simulink library "outp"  (R2021b)
(part 6 of 7)

  VTPM_S4ID_raw32_Inproc : FVT_lib/outp/OverrideAndLimit  SystemSampleTime=-1  VariantActivationTime=update diagram  Latency=0  AutoFrameSizeCalculation=off
      link override Signal_Limit/_maxval: Value=KOUTP_S4ID_raw32_maxval
      link override Signal_Limit/_minval: Value=KOUTP_S4ID_raw32_minval
      link override Signal_Override/_ovrdflg: Value=KOUTP_S4ID_raw32_ovrdflg
      link override Signal_Override/_ovrdval: Value=KOUTP_S4ID_raw32_ovrdval
  VTPM_S4L_enum_Inproc : FVT_lib/outp/OverrideAndLimit  SystemSampleTime=-1  VariantActivationTime=update diagram  Latency=0  AutoFrameSizeCalculation=off
      link override Signal_Limit/_maxval: Value=KOUTP_S4L_enum_maxval
      link override Signal_Limit/_minval: Value=KOUTP_S4L_enum_minval
      link override Signal_Override/_ovrdflg: Value=KOUTP_S4L_enum_ovrdflg
      link override Signal_Override/_ovrdval: Value=KOUTP_S4L_enum_ovrdval
  VTPM_S4WheelDebugALTU_pct_Inproc : FVT_lib/outp/OverrideAndLimit  SystemSampleTime=-1  VariantActivationTime=update diagram  Latency=0  AutoFrameSizeCalculation=off
      link override Signal_Limit/_maxval: Value=KOUTP_S4WheelDebugALTU_pct_maxval
      link override Signal_Limit/_minval: Value=KOUTP_S4WheelDebugALTU_pct_minval
      link override Signal_Override/_ovrdflg: Value=KOUTP_S4WheelDebugALTU_pct_ovrdflg
      link override Signal_Override/_ovrdval: Value=KOUTP_S4WheelDebugALTU_pct_ovrdval
  VTPM_SetIDLoc_flg_Inproc : FVT_lib/outp/OverrideAndLimit  SystemSampleTime=-1  VariantActivationTime=update diagram  Latency=0  AutoFrameSizeCalculation=off
      link override Signal_Limit/_maxval: Value=KOUTP_SetIDLoc_flg_maxval
      link override Signal_Limit/_minval: Value=KOUTP_SetIDLoc_flg_minval
      link override Signal_Override/_ovrdflg: Value=KOUTP_SetIDLoc_flg_ovrdflg
      link override Signal_Override/_ovrdval: Value=KOUTP_SetIDLoc_flg_ovrdval
  VTPM_TPMSCaliButtAllow_flg_Inproc : FVT_lib/outp/OverrideAndLimit  SystemSampleTime=-1  VariantActivationTime=update diagram  Latency=0  AutoFrameSizeCalculation=off
      link override Signal_Limit/_maxval: Value=KOUTP_TPMSCaliButtAllow_flg_maxval
      link override Signal_Limit/_minval: Value=KOUTP_TPMSCaliButtAllow_flg_minval
      link override Signal_Override/_ovrdflg: Value=KOUTP_TPMSCaliButtAllow_flg_ovrdflg
      link override Signal_Override/_ovrdval: Value=KOUTP_TPMSCaliButtAllow_flg_ovrdval
  VTPM_TPMSResButtAllow_flg_Inproc : FVT_lib/outp/OverrideAndLimit  SystemSampleTime=-1  VariantActivationTime=update diagram  Latency=0  AutoFrameSizeCalculation=off
      link override Signal_Limit/_maxval: Value=KOUTP_TPMSResButtAllow_flg_maxval
      link override Signal_Limit/_minval: Value=KOUTP_TPMSResButtAllow_flg_minval
      link override Signal_Override/_ovrdflg: Value=KOUTP_TPMSResButtAllow_flg_ovrdflg
      link override Signal_Override/_ovrdval: Value=KOUTP_TPMSResButtAllow_flg_ovrdval
  VTPM_TPMSResButt_flg_Inproc : FVT_lib/outp/OverrideAndLimit  SystemSampleTime=-1  VariantActivationTime=update diagram  Latency=0  AutoFrameSizeCalculation=off
      link override Signal_Limit/_maxval: Value=KOUTP_TPMSResButt_flg_maxval
      link override Signal_Limit/_minval: Value=KOUTP_TPMSResButt_flg_minval
      link override Signal_Override/_ovrdflg: Value=KOUTP_TPMSResButt_flg_ovrdflg
      link override Signal_Override/_ovrdval: Value=KOUTP_TPMSResButt_flg_ovrdval
  VTPM_TPMSStorge_flg_Inproc : FVT_lib/outp/OverrideAndLimit  SystemSampleTime=-1  VariantActivationTime=update diagram  Latency=0  AutoFrameSizeCalculation=off
      link override Signal_Limit/_maxval: Value=KOUTP_TPMSStorge_flg_maxval
      link override Signal_Limit/_minval: Value=KOUTP_TPMSStorge_flg_minval
      link override Signal_Override/_ovrdflg: Value=KOUTP_TPMSStorge_flg_ovrdflg
      link override Signal_Override/_ovrdval: Value=KOUTP_TPMSStorge_flg_ovrdval
  VTPM_TPMSWarnIndi_enum_Inproc : FVT_lib/outp/OverrideAndLimit  SystemSampleTime=-1  VariantActivationTime=update diagram  Latency=0  AutoFrameSizeCalculation=off
      link override Signal_Limit/_maxval: Value=KOUTP_TPMSWarnIndi_enum_maxval
      link override Signal_Limit/_minval: Value=KOUTP_TPMSWarnIndi_enum_minval
      link override Signal_Override/_ovrdflg: Value=KOUTP_TPMSWarnIndi_enum_ovrdflg
      link override Signal_Override/_ovrdval: Value=KOUTP_TPMSWarnIndi_enum_ovrdval
  VTPM_WriteChkLFID_raw_Inproc : FVT_lib/outp/OverrideAndLimit  SystemSampleTime=-1  VariantActivationTime=update diagram  Latency=0  AutoFrameSizeCalculation=off
      link override Signal_Limit/_maxval: Value=KOUTP_WriteChkLFID_raw_maxval
      link override Signal_Limit/_minval: Value=KOUTP_WriteChkLFID_raw_minval
      link override Signal_Override/_ovrdflg: Value=KOUTP_WriteChkLFID_raw_ovrdflg
      link override Signal_Override/_ovrdval: Value=KOUTP_WriteChkLFID_raw_ovrdval
  VTPM_WriteChkLRID_raw_Inproc : FVT_lib/outp/OverrideAndLimit  SystemSampleTime=-1  VariantActivationTime=update diagram  Latency=0  AutoFrameSizeCalculation=off
      link override Signal_Limit/_maxval: Value=KOUTP_WriteChkLRID_raw_maxval
      link override Signal_Limit/_minval: Value=KOUTP_WriteChkLRID_raw_minval
      link override Signal_Override/_ovrdflg: Value=KOUTP_WriteChkLRID_raw_ovrdflg
      link override Signal_Override/_ovrdval: Value=KOUTP_WriteChkLRID_raw_ovrdval
  VTPM_WriteChkRFID_raw_Inproc : FVT_lib/outp/OverrideAndLimit  SystemSampleTime=-1  VariantActivationTime=update diagram  Latency=0  AutoFrameSizeCalculation=off
      link override Signal_Limit/_maxval: Value=KOUTP_WriteChkRFID_raw_maxval
      link override Signal_Limit/_minval: Value=KOUTP_WriteChkRFID_raw_minval
      link override Signal_Override/_ovrdflg: Value=KOUTP_WriteChkRFID_raw_ovrdflg
      link override Signal_Override/_ovrdval: Value=KOUTP_WriteChkRFID_raw_ovrdval
  VTPM_WriteChkRRID_raw_Inproc : FVT_lib/outp/OverrideAndLimit  SystemSampleTime=-1  VariantActivationTime=update diagram  Latency=0  AutoFrameSizeCalculation=off
      link override Signal_Limit/_maxval: Value=KOUTP_WriteChkRRID_raw_maxval
      link override Signal_Limit/_minval: Value=KOUTP_WriteChkRRID_raw_minval
      link override Signal_Override/_ovrdflg: Value=KOUTP_WriteChkRRID_raw_ovrdflg
      link override Signal_Override/_ovrdval: Value=KOUTP_WriteChkRRID_raw_ovrdval
  VTPM_WriteChkfinLFID_raw_Inproc : FVT_lib/outp/OverrideAndLimit  SystemSampleTime=-1  VariantActivationTime=update diagram  Latency=0  AutoFrameSizeCalculation=off
      link override Signal_Limit/_maxval: Value=KOUTP_WriteChkfinLFID_raw_maxval
      link override Signal_Limit/_minval: Value=KOUTP_WriteChkfinLFID_raw_minval
      link override Signal_Override/_ovrdflg: Value=KOUTP_WriteChkfinLFID_raw_ovrdflg
      link override Signal_Override/_ovrdval: Value=KOUTP_WriteChkfinLFID_raw_ovrdval
  VTPM_WriteChkfinLRID_raw_Inproc : FVT_lib/outp/OverrideAndLimit  SystemSampleTime=-1  VariantActivationTime=update diagram  Latency=0  AutoFrameSizeCalculation=off
      link override Signal_Limit/_maxval: Value=KOUTP_WriteChkfinLRID_raw_maxval
      link override Signal_Limit/_minval: Value=KOUTP_WriteChkfinLRID_raw_minval
      link override Signal_Override/_ovrdflg: Value=KOUTP_WriteChkfinLRID_raw_ovrdflg
      link override Signal_Override/_ovrdval: Value=KOUTP_WriteChkfinLRID_raw_ovrdval
  VTPM_WriteChkfinRFID_raw_Inproc : FVT_lib/outp/OverrideAndLimit  SystemSampleTime=-1  VariantActivationTime=update diagram  Latency=0  AutoFrameSizeCalculation=off
      link override Signal_Limit/_maxval: Value=KOUTP_WriteChkfinRFID_raw_maxval
      link override Signal_Limit/_minval: Value=KOUTP_WriteChkfinRFID_raw_minval
      link override Signal_Override/_ovrdflg: Value=KOUTP_WriteChkfinRFID_raw_ovrdflg
      link override Signal_Override/_ovrdval: Value=KOUTP_WriteChkfinRFID_raw_ovrdval
  VTPM_WriteChkfinRRID_raw_Inproc : FVT_lib/outp/OverrideAndLimit  SystemSampleTime=-1  VariantActivationTime=update diagram  Latency=0  AutoFrameSizeCalculation=off
      link override Signal_Limit/_maxval: Value=KOUTP_WriteChkfinRRID_raw_maxval
      link override Signal_Limit/_minval: Value=KOUTP_WriteChkfinRRID_raw_minval
      link override Signal_Override/_ovrdflg: Value=KOUTP_WriteChkfinRRID_raw_ovrdflg
      link override Signal_Override/_ovrdval: Value=KOUTP_WriteChkfinRRID_raw_ovrdval
  VTPM_unlearnSfailvalid_enum_Inproc : FVT_lib/outp/OverrideAndLimit  SystemSampleTime=-1  VariantActivationTime=update diagram  Latency=0  AutoFrameSizeCalculation=off
      link override Signal_Limit/_maxval: Value=KOUTP_unlearnSfailvalid_enum_maxval
      link override Signal_Limit/_minval: Value=KOUTP_unlearnSfailvalid_enum_minval
      link override Signal_Override/_ovrdflg: Value=KOUTP_unlearnSfailvalid_enum_ovrdflg
      link override Signal_Override/_ovrdval: Value=KOUTP_unlearnSfailvalid_enum_ovrdval
  VTPM_unlearnSfali_flg_Inproc : FVT_lib/outp/OverrideAndLimit  SystemSampleTime=-1  VariantActivationTime=update diagram  Latency=0  AutoFrameSizeCalculation=off
      link override Signal_Limit/_maxval: Value=KOUTP_unlearnSfali_flg_maxval
      link override Signal_Limit/_minval: Value=KOUTP_unlearnSfali_flg_minval
      link override Signal_Override/_ovrdflg: Value=KOUTP_unlearnSfali_flg_ovrdflg
      link override Signal_Override/_ovrdval: Value=KOUTP_unlearnSfali_flg_ovrdval
  VTQD_ActParkRequest_flg_Inproc : FVT_lib/outp/OverrideAndLimit  SystemSampleTime=-1  VariantActivationTime=update diagram  Latency=0  AutoFrameSizeCalculation=off
      link override Signal_Limit/_maxval: Value=KOUTP_ActParkRequest_flg_maxval
      link override Signal_Limit/_minval: Value=KOUTP_ActParkRequest_flg_minval
      link override Signal_Override/_ovrdflg: Value=KOUTP_ActParkRequest_flg_ovrdflg
      link override Signal_Override/_ovrdval: Value=KOUTP_ActParkRequest_flg_ovrdval
  VTQD_CreepON_flg_Inproc : FVT_lib/outp/OverrideAndLimit  SystemSampleTime=-1  VariantActivationTime=update diagram  Latency=0  AutoFrameSizeCalculation=off
      link override Signal_Limit/_maxval: Value=KOUTP_CreepON_flg_maxval
      link override Signal_Limit/_minval: Value=KOUTP_CreepON_flg_minval
      link override Signal_Override/_ovrdflg: Value=KOUTP_CreepON_flg_ovrdflg
      link override Signal_Override/_ovrdval: Value=KOUTP_CreepON_flg_ovrdval
  VTQD_DriveProtEn_flg_Inproc : FVT_lib/outp/OverrideAndLimit  SystemSampleTime=-1  VariantActivationTime=update diagram  Latency=0  AutoFrameSizeCalculation=off
      link override Signal_Limit/_maxval: Value=KOUTP_DriveProtEn_flg_maxval
      link override Signal_Limit/_minval: Value=KOUTP_DriveProtEn_flg_minval
      link override Signal_Override/_ovrdflg: Value=KOUTP_DriveProtEn_flg_ovrdflg
      link override Signal_Override/_ovrdval: Value=KOUTP_DriveProtEn_flg_ovrdval
  VTQD_DriverWhlTqDemFr_Nm_Inproc : FVT_lib/outp/OverrideAndLimit  SystemSampleTime=-1  VariantActivationTime=update diagram  Latency=0  AutoFrameSizeCalculation=off
      link override Signal_Limit/_maxval: Value=KOUTP_DriverWhlTqDemFr_Nm_maxval
      link override Signal_Limit/_minval: Value=KOUTP_DriverWhlTqDemFr_Nm_minval
      link override Signal_Override/_ovrdflg: Value=KOUTP_DriverWhlTqDemFr_Nm_ovrdflg
      link override Signal_Override/_ovrdval: Value=KOUTP_DriverWhlTqDemFr_Nm_ovrdval
  VTQD_DriverWhlTqDemRr_Nm_Inproc : FVT_lib/outp/OverrideAndLimit  SystemSampleTime=-1  VariantActivationTime=update diagram  Latency=0  AutoFrameSizeCalculation=off
      link override Signal_Limit/_maxval: Value=KOUTP_DriverWhlTqDemRr_Nm_maxval
      link override Signal_Limit/_minval: Value=KOUTP_DriverWhlTqDemRr_Nm_minval
      link override Signal_Override/_ovrdflg: Value=KOUTP_DriverWhlTqDemRr_Nm_ovrdflg
      link override Signal_Override/_ovrdval: Value=KOUTP_DriverWhlTqDemRr_Nm_ovrdval
  VTQD_EVDriveMode_enum_Inproc : FVT_lib/outp/OverrideAndLimit  SystemSampleTime=-1  VariantActivationTime=update diagram  Latency=0  AutoFrameSizeCalculation=off
      link override Signal_Limit/_maxval: Value=KOUTP_EVDriveMode_enum_maxval
      link override Signal_Limit/_minval: Value=KOUTP_EVDriveMode_enum_minval
      link override Signal_Override/_ovrdflg: Value=KOUTP_EVDriveMode_enum_ovrdflg
      link override Signal_Override/_ovrdval: Value=KOUTP_EVDriveMode_enum_ovrdval
  VTQD_EquivAccPedalSWSta_flg_Inproc : FVT_lib/outp/OverrideAndLimit  SystemSampleTime=-1  VariantActivationTime=update diagram  Latency=0  AutoFrameSizeCalculation=off
      link override Signal_Limit/_maxval: Value=KOUTP_EquivAccPedalSWSta_flg_maxval
      link override Signal_Limit/_minval: Value=KOUTP_EquivAccPedalSWSta_flg_minval
      link override Signal_Override/_ovrdflg: Value=KOUTP_EquivAccPedalSWSta_flg_ovrdflg
      link override Signal_Override/_ovrdval: Value=KOUTP_EquivAccPedalSWSta_flg_ovrdval
  VTQD_FDCVCURegenMode_enum_Inproc : FVT_lib/outp/OverrideAndLimit  SystemSampleTime=-1  VariantActivationTime=update diagram  Latency=0  AutoFrameSizeCalculation=off
      link override Signal_Limit/_maxval: Value=KOUTP_FDCVCURegenMode_enum_maxval
      link override Signal_Limit/_minval: Value=KOUTP_FDCVCURegenMode_enum_minval
      link override Signal_Override/_ovrdflg: Value=KOUTP_FDCVCURegenMode_enum_ovrdflg
      link override Signal_Override/_ovrdval: Value=KOUTP_FDCVCURegenMode_enum_ovrdval
  VTQD_FrActvDmpDisabReq_flg_Inproc : FVT_lib/outp/OverrideAndLimit  SystemSampleTime=-1  VariantActivationTime=update diagram  Latency=0  AutoFrameSizeCalculation=off
      link override Signal_Limit/_maxval: Value=KOUTP_FrActvDmpDisabReq_flg_maxval
      link override Signal_Limit/_minval: Value=KOUTP_FrActvDmpDisabReq_flg_minval
      link override Signal_Override/_ovrdflg: Value=KOUTP_FrActvDmpDisabReq_flg_ovrdflg
      link override Signal_Override/_ovrdval: Value=KOUTP_FrActvDmpDisabReq_flg_ovrdval
  VTQD_FrEDUActTq_Nm_Inproc : FVT_lib/outp/OverrideAndLimit  SystemSampleTime=-1  VariantActivationTime=update diagram  Latency=0  AutoFrameSizeCalculation=off
      link override Signal_Limit/_maxval: Value=KOUTP_FrEDUActTq_Nm_maxval
      link override Signal_Limit/_minval: Value=KOUTP_FrEDUActTq_Nm_minval
      link override Signal_Override/_ovrdflg: Value=KOUTP_FrEDUActTq_Nm_ovrdflg
      link override Signal_Override/_ovrdval: Value=KOUTP_FrEDUActTq_Nm_ovrdval
  VTQD_FrEDUAvailBrkRgnTqV_flg_Inproc : FVT_lib/outp/OverrideAndLimit  SystemSampleTime=-1  VariantActivationTime=update diagram  Latency=0  AutoFrameSizeCalculation=off
      link override Signal_Limit/_maxval: Value=KOUTP_FrEDUAvailBrkRgnTqV_flg_maxval
      link override Signal_Limit/_minval: Value=KOUTP_FrEDUAvailBrkRgnTqV_flg_minval
      link override Signal_Override/_ovrdflg: Value=KOUTP_FrEDUAvailBrkRgnTqV_flg_ovrdflg
      link override Signal_Override/_ovrdval: Value=KOUTP_FrEDUAvailBrkRgnTqV_flg_ovrdval
  VTQD_FrEDUAvailBrkRgnTq_Nm_Inproc : FVT_lib/outp/OverrideAndLimit  SystemSampleTime=-1  VariantActivationTime=update diagram  Latency=0  AutoFrameSizeCalculation=off
      link override Signal_Limit/_maxval: Value=KOUTP_FrEDUAvailBrkRgnTq_Nm_maxval
      link override Signal_Limit/_minval: Value=KOUTP_FrEDUAvailBrkRgnTq_Nm_minval
      link override Signal_Override/_ovrdflg: Value=KOUTP_FrEDUAvailBrkRgnTq_Nm_ovrdflg
      link override Signal_Override/_ovrdval: Value=KOUTP_FrEDUAvailBrkRgnTq_Nm_ovrdval
  VTQD_FrEDURolRgnTq_Nm_Inproc : FVT_lib/outp/OverrideAndLimit  SystemSampleTime=-1  VariantActivationTime=update diagram  Latency=0  AutoFrameSizeCalculation=off
      link override Signal_Limit/_maxval: Value=KOUTP_FrEDURolRgnTq_Nm_maxval
      link override Signal_Limit/_minval: Value=KOUTP_FrEDURolRgnTq_Nm_minval
      link override Signal_Override/_ovrdflg: Value=KOUTP_FrEDURolRgnTq_Nm_ovrdflg
      link override Signal_Override/_ovrdval: Value=KOUTP_FrEDURolRgnTq_Nm_ovrdval
  VTQD_FrEDUSpdValid_flg_Inproc : FVT_lib/outp/OverrideAndLimit  SystemSampleTime=-1  VariantActivationTime=update diagram  Latency=0  AutoFrameSizeCalculation=off
      link override Signal_Limit/_maxval: Value=KOUTP_FrEDUSpdValid_flg_maxval
      link override Signal_Limit/_minval: Value=KOUTP_FrEDUSpdValid_flg_minval
      link override Signal_Override/_ovrdflg: Value=KOUTP_FrEDUSpdValid_flg_ovrdflg
      link override Signal_Override/_ovrdval: Value=KOUTP_FrEDUSpdValid_flg_ovrdval
  VTQD_FrEDUSpd_rpm_Inproc : FVT_lib/outp/OverrideAndLimit  SystemSampleTime=-1  VariantActivationTime=update diagram  Latency=0  AutoFrameSizeCalculation=off
      link override Signal_Limit/_maxval: Value=KOUTP_FrEDUSpd_rpm_maxval
      link override Signal_Limit/_minval: Value=KOUTP_FrEDUSpd_rpm_minval
      link override Signal_Override/_ovrdflg: Value=KOUTP_FrEDUSpd_rpm_ovrdflg
      link override Signal_Override/_ovrdval: Value=KOUTP_FrEDUSpd_rpm_ovrdval
  VTQD_FrIdcMax_A_Inproc : FVT_lib/outp/OverrideAndLimit  SystemSampleTime=-1  VariantActivationTime=update diagram  Latency=0  AutoFrameSizeCalculation=off
      link override Signal_Limit/_maxval: Value=KOUTP_FrIdcMax_A_maxval
      link override Signal_Limit/_minval: Value=KOUTP_FrIdcMax_A_minval
      link override Signal_Override/_ovrdflg: Value=KOUTP_FrIdcMax_A_ovrdflg
      link override Signal_Override/_ovrdval: Value=KOUTP_FrIdcMax_A_ovrdval
  VTQD_FrIdcMin_A_Inproc : FVT_lib/outp/OverrideAndLimit  SystemSampleTime=-1  VariantActivationTime=update diagram  Latency=0  AutoFrameSizeCalculation=off
      link override Signal_Limit/_maxval: Value=KOUTP_FrIdcMin_A_maxval
      link override Signal_Limit/_minval: Value=KOUTP_FrIdcMin_A_minval
      link override Signal_Override/_ovrdflg: Value=KOUTP_FrIdcMin_A_ovrdflg
      link override Signal_Override/_ovrdval: Value=KOUTP_FrIdcMin_A_ovrdval
  VTQD_FrRgnDecrSta_flg_Inproc : FVT_lib/outp/OverrideAndLimit  SystemSampleTime=-1  VariantActivationTime=update diagram  Latency=0  AutoFrameSizeCalculation=off
      link override Signal_Limit/_maxval: Value=KOUTP_FrRgnDecrSta_flg_maxval
      link override Signal_Limit/_minval: Value=KOUTP_FrRgnDecrSta_flg_minval
      link override Signal_Override/_ovrdflg: Value=KOUTP_FrRgnDecrSta_flg_ovrdflg
      link override Signal_Override/_ovrdval: Value=KOUTP_FrRgnDecrSta_flg_ovrdval
  VTQD_FrRgnPermSta_flg_Inproc : FVT_lib/outp/OverrideAndLimit  SystemSampleTime=-1  VariantActivationTime=update diagram  Latency=0  AutoFrameSizeCalculation=off
      link override Signal_Limit/_maxval: Value=KOUTP_FrRgnPermSta_flg_maxval
      link override Signal_Limit/_minval: Value=KOUTP_FrRgnPermSta_flg_minval
      link override Signal_Override/_ovrdflg: Value=KOUTP_FrRgnPermSta_flg_ovrdflg
      link override Signal_Override/_ovrdval: Value=KOUTP_FrRgnPermSta_flg_ovrdval
  VTQD_FrUdcMax_V_Inproc : FVT_lib/outp/OverrideAndLimit  SystemSampleTime=-1  VariantActivationTime=update diagram  Latency=0  AutoFrameSizeCalculation=off
      link override Signal_Limit/_maxval: Value=KOUTP_FrUdcMax_V_maxval
      link override Signal_Limit/_minval: Value=KOUTP_FrUdcMax_V_minval
      link override Signal_Override/_ovrdflg: Value=KOUTP_FrUdcMax_V_ovrdflg
      link override Signal_Override/_ovrdval: Value=KOUTP_FrUdcMax_V_ovrdval
  VTQD_FrUdcMin_V_Inproc : FVT_lib/outp/OverrideAndLimit  SystemSampleTime=-1  VariantActivationTime=update diagram  Latency=0  AutoFrameSizeCalculation=off
      link override Signal_Limit/_maxval: Value=KOUTP_FrUdcMin_V_maxval
      link override Signal_Limit/_minval: Value=KOUTP_FrUdcMin_V_minval
      link override Signal_Override/_ovrdflg: Value=KOUTP_FrUdcMin_V_ovrdflg
      link override Signal_Override/_ovrdval: Value=KOUTP_FrUdcMin_V_ovrdval
  VTQD_IVIPwrLockSta_enum_Inproc : FVT_lib/outp/OverrideAndLimit  SystemSampleTime=-1  VariantActivationTime=update diagram  Latency=0  AutoFrameSizeCalculation=off
      link override Signal_Limit/_maxval: Value=KOUTP_IVIPwrLockSta_enum_maxval
      link override Signal_Limit/_minval: Value=KOUTP_IVIPwrLockSta_enum_minval
      link override Signal_Override/_ovrdflg: Value=KOUTP_IVIPwrLockSta_enum_ovrdflg
      link override Signal_Override/_ovrdval: Value=KOUTP_IVIPwrLockSta_enum_ovrdval
  VTQD_OPDHoldLamp_flg_Inproc : FVT_lib/outp/OverrideAndLimit  SystemSampleTime=-1  VariantActivationTime=update diagram  Latency=0  AutoFrameSizeCalculation=off
      link override Signal_Limit/_maxval: Value=KOUTP_OPDHoldLamp_flg_maxval
      link override Signal_Limit/_minval: Value=KOUTP_OPDHoldLamp_flg_minval
      link override Signal_Override/_ovrdflg: Value=KOUTP_OPDHoldLamp_flg_ovrdflg
      link override Signal_Override/_ovrdval: Value=KOUTP_OPDHoldLamp_flg_ovrdval
  VTQD_PButtonSta_enum_Inproc : FVT_lib/outp/OverrideAndLimit  SystemSampleTime=-1  VariantActivationTime=update diagram  Latency=0  AutoFrameSizeCalculation=off
      link override Signal_Limit/_maxval: Value=KOUTP_PButtonSta_enum_maxval
      link override Signal_Limit/_minval: Value=KOUTP_PButtonSta_enum_minval
      link override Signal_Override/_ovrdflg: Value=KOUTP_PButtonSta_enum_ovrdflg
      link override Signal_Override/_ovrdval: Value=KOUTP_PButtonSta_enum_ovrdval
  VTQD_PTCSPermSta_flg_Inproc : FVT_lib/outp/OverrideAndLimit  SystemSampleTime=-1  VariantActivationTime=update diagram  Latency=0  AutoFrameSizeCalculation=off
      link override Signal_Limit/_maxval: Value=KOUTP_PTCSPermSta_flg_maxval
      link override Signal_Limit/_minval: Value=KOUTP_PTCSPermSta_flg_minval
      link override Signal_Override/_ovrdflg: Value=KOUTP_PTCSPermSta_flg_ovrdflg
      link override Signal_Override/_ovrdval: Value=KOUTP_PTCSPermSta_flg_ovrdval
  VTQD_ParkRequest_flg_Inproc : FVT_lib/outp/OverrideAndLimit  SystemSampleTime=-1  VariantActivationTime=update diagram  Latency=0  AutoFrameSizeCalculation=off
      link override Signal_Limit/_maxval: Value=KOUTP_ParkRequest_flg_maxval
      link override Signal_Limit/_minval: Value=KOUTP_ParkRequest_flg_minval
      link override Signal_Override/_ovrdflg: Value=KOUTP_ParkRequest_flg_ovrdflg
      link override Signal_Override/_ovrdval: Value=KOUTP_ParkRequest_flg_ovrdval
  VTQD_ReBrakeLPReq_flg_Inproc : FVT_lib/outp/OverrideAndLimit  SystemSampleTime=-1  VariantActivationTime=update diagram  Latency=0  AutoFrameSizeCalculation=off
      link override Signal_Limit/_maxval: Value=KOUTP_ReBrakeLPReq_flg_maxval
      link override Signal_Limit/_minval: Value=KOUTP_ReBrakeLPReq_flg_minval
      link override Signal_Override/_ovrdflg: Value=KOUTP_ReBrakeLPReq_flg_ovrdflg
      link override Signal_Override/_ovrdval: Value=KOUTP_ReBrakeLPReq_flg_ovrdval
  VTQD_RgnAbnorSta_flg_Inproc : FVT_lib/outp/OverrideAndLimit  SystemSampleTime=-1  VariantActivationTime=update diagram  Latency=0  AutoFrameSizeCalculation=off
      link override Signal_Limit/_maxval: Value=KOUTP_RgnAbnorSta_flg_maxval
      link override Signal_Limit/_minval: Value=KOUTP_RgnAbnorSta_flg_minval
      link override Signal_Override/_ovrdflg: Value=KOUTP_RgnAbnorSta_flg_ovrdflg
      link override Signal_Override/_ovrdval: Value=KOUTP_RgnAbnorSta_flg_ovrdval
  VTQD_RrActvDmpDisabReq_flg_Inproc : FVT_lib/outp/OverrideAndLimit  SystemSampleTime=-1  VariantActivationTime=update diagram  Latency=0  AutoFrameSizeCalculation=off
      link override Signal_Limit/_maxval: Value=KOUTP_RrActvDmpDisabReq_flg_maxval
      link override Signal_Limit/_minval: Value=KOUTP_RrActvDmpDisabReq_flg_minval
      link override Signal_Override/_ovrdflg: Value=KOUTP_RrActvDmpDisabReq_flg_ovrdflg
      link override Signal_Override/_ovrdval: Value=KOUTP_RrActvDmpDisabReq_flg_ovrdval
  VTQD_RrEDUActTq_Nm_Inproc : FVT_lib/outp/OverrideAndLimit  SystemSampleTime=-1  VariantActivationTime=update diagram  Latency=0  AutoFrameSizeCalculation=off
      link override Signal_Limit/_maxval: Value=KOUTP_RrEDUActTq_Nm_maxval
      link override Signal_Limit/_minval: Value=KOUTP_RrEDUActTq_Nm_minval
      link override Signal_Override/_ovrdflg: Value=KOUTP_RrEDUActTq_Nm_ovrdflg
      link override Signal_Override/_ovrdval: Value=KOUTP_RrEDUActTq_Nm_ovrdval
  VTQD_RrEDUAvailBrkRgnTqV_flg_Inproc : FVT_lib/outp/OverrideAndLimit  SystemSampleTime=-1  VariantActivationTime=update diagram  Latency=0  AutoFrameSizeCalculation=off
      link override Signal_Limit/_maxval: Value=KOUTP_RrEDUAvailBrkRgnTqV_flg_maxval
      link override Signal_Limit/_minval: Value=KOUTP_RrEDUAvailBrkRgnTqV_flg_minval
      link override Signal_Override/_ovrdflg: Value=KOUTP_RrEDUAvailBrkRgnTqV_flg_ovrdflg
      link override Signal_Override/_ovrdval: Value=KOUTP_RrEDUAvailBrkRgnTqV_flg_ovrdval
  VTQD_RrEDUAvailBrkRgnTq_Nm_Inproc : FVT_lib/outp/OverrideAndLimit  SystemSampleTime=-1  VariantActivationTime=update diagram  Latency=0  AutoFrameSizeCalculation=off
      link override Signal_Limit/_maxval: Value=KOUTP_RrEDUAvailBrkRgnTq_Nm_maxval
      link override Signal_Limit/_minval: Value=KOUTP_RrEDUAvailBrkRgnTq_Nm_minval
      link override Signal_Override/_ovrdflg: Value=KOUTP_RrEDUAvailBrkRgnTq_Nm_ovrdflg
      link override Signal_Override/_ovrdval: Value=KOUTP_RrEDUAvailBrkRgnTq_Nm_ovrdval
  VTQD_RrEDURolRgnTq_Nm_Inproc : FVT_lib/outp/OverrideAndLimit  SystemSampleTime=-1  VariantActivationTime=update diagram  Latency=0  AutoFrameSizeCalculation=off
      link override Signal_Limit/_maxval: Value=KOUTP_RrEDURolRgnTq_Nm_maxval
      link override Signal_Limit/_minval: Value=KOUTP_RrEDURolRgnTq_Nm_minval
      link override Signal_Override/_ovrdflg: Value=KOUTP_RrEDURolRgnTq_Nm_ovrdflg
      link override Signal_Override/_ovrdval: Value=KOUTP_RrEDURolRgnTq_Nm_ovrdval
  VTQD_RrEDUSpdValid_flg_Inproc : FVT_lib/outp/OverrideAndLimit  SystemSampleTime=-1  VariantActivationTime=update diagram  Latency=0  AutoFrameSizeCalculation=off
      link override Signal_Limit/_maxval: Value=KOUTP_RrEDUSpdValid_flg_maxval
      link override Signal_Limit/_minval: Value=KOUTP_RrEDUSpdValid_flg_minval
      link override Signal_Override/_ovrdflg: Value=KOUTP_RrEDUSpdValid_flg_ovrdflg
      link override Signal_Override/_ovrdval: Value=KOUTP_RrEDUSpdValid_flg_ovrdval
  VTQD_RrEDUSpd_rpm_Inproc : FVT_lib/outp/OverrideAndLimit  SystemSampleTime=-1  VariantActivationTime=update diagram  Latency=0  AutoFrameSizeCalculation=off
      link override Signal_Limit/_maxval: Value=KOUTP_RrEDUSpd_rpm_maxval
      link override Signal_Limit/_minval: Value=KOUTP_RrEDUSpd_rpm_minval
      link override Signal_Override/_ovrdflg: Value=KOUTP_RrEDUSpd_rpm_ovrdflg
      link override Signal_Override/_ovrdval: Value=KOUTP_RrEDUSpd_rpm_ovrdval
  VTQD_RrIdcMax_A_Inproc : FVT_lib/outp/OverrideAndLimit  SystemSampleTime=-1  VariantActivationTime=update diagram  Latency=0  AutoFrameSizeCalculation=off
      link override Signal_Limit/_maxval: Value=KOUTP_RrIdcMax_A_maxval
      link override Signal_Limit/_minval: Value=KOUTP_RrIdcMax_A_minval
      link override Signal_Override/_ovrdflg: Value=KOUTP_RrIdcMax_A_ovrdflg
      link override Signal_Override/_ovrdval: Value=KOUTP_RrIdcMax_A_ovrdval
  VTQD_RrIdcMin_A_Inproc : FVT_lib/outp/OverrideAndLimit  SystemSampleTime=-1  VariantActivationTime=update diagram  Latency=0  AutoFrameSizeCalculation=off
      link override Signal_Limit/_maxval: Value=KOUTP_RrIdcMin_A_maxval
      link override Signal_Limit/_minval: Value=KOUTP_RrIdcMin_A_minval
      link override Signal_Override/_ovrdflg: Value=KOUTP_RrIdcMin_A_ovrdflg
      link override Signal_Override/_ovrdval: Value=KOUTP_RrIdcMin_A_ovrdval
  VTQD_RrRgnDecrSta_flg_Inproc : FVT_lib/outp/OverrideAndLimit  SystemSampleTime=-1  VariantActivationTime=update diagram  Latency=0  AutoFrameSizeCalculation=off
      link override Signal_Limit/_maxval: Value=KOUTP_RrRgnDecrSta_flg_maxval
      link override Signal_Limit/_minval: Value=KOUTP_RrRgnDecrSta_flg_minval
      link override Signal_Override/_ovrdflg: Value=KOUTP_RrRgnDecrSta_flg_ovrdflg
      link override Signal_Override/_ovrdval: Value=KOUTP_RrRgnDecrSta_flg_ovrdval
  VTQD_RrRgnPermSta_flg_Inproc : FVT_lib/outp/OverrideAndLimit  SystemSampleTime=-1  VariantActivationTime=update diagram  Latency=0  AutoFrameSizeCalculation=off
      link override Signal_Limit/_maxval: Value=KOUTP_RrRgnPermSta_flg_maxval
      link override Signal_Limit/_minval: Value=KOUTP_RrRgnPermSta_flg_minval
      link override Signal_Override/_ovrdflg: Value=KOUTP_RrRgnPermSta_flg_ovrdflg
      link override Signal_Override/_ovrdval: Value=KOUTP_RrRgnPermSta_flg_ovrdval
  VTQD_RrUdcMax_V_Inproc : FVT_lib/outp/OverrideAndLimit  SystemSampleTime=-1  VariantActivationTime=update diagram  Latency=0  AutoFrameSizeCalculation=off
      link override Signal_Limit/_maxval: Value=KOUTP_RrUdcMax_V_maxval
      link override Signal_Limit/_minval: Value=KOUTP_RrUdcMax_V_minval
      link override Signal_Override/_ovrdflg: Value=KOUTP_RrUdcMax_V_ovrdflg
      link override Signal_Override/_ovrdval: Value=KOUTP_RrUdcMax_V_ovrdval
  VTQD_RrUdcMin_V_Inproc : FVT_lib/outp/OverrideAndLimit  SystemSampleTime=-1  VariantActivationTime=update diagram  Latency=0  AutoFrameSizeCalculation=off
      link override Signal_Limit/_maxval: Value=KOUTP_RrUdcMin_V_maxval
      link override Signal_Limit/_minval: Value=KOUTP_RrUdcMin_V_minval
      link override Signal_Override/_ovrdflg: Value=KOUTP_RrUdcMin_V_ovrdflg
      link override Signal_Override/_ovrdval: Value=KOUTP_RrUdcMin_V_ovrdval
  VTQD_SaveRegenMode_enum_Inproc : FVT_lib/outp/OverrideAndLimit  SystemSampleTime=-1  VariantActivationTime=update diagram  Latency=0  AutoFrameSizeCalculation=off
      link override Signal_Limit/_maxval: Value=KOUTP_SaveRegenMode_enum_maxval
      link override Signal_Limit/_minval: Value=KOUTP_SaveRegenMode_enum_minval
      link override Signal_Override/_ovrdflg: Value=KOUTP_SaveRegenMode_enum_ovrdflg
      link override Signal_Override/_ovrdval: Value=KOUTP_SaveRegenMode_enum_ovrdval
  VTQD_SetSpd_kph_Inproc : FVT_lib/outp/OverrideAndLimit  SystemSampleTime=-1  VariantActivationTime=update diagram  Latency=0  AutoFrameSizeCalculation=off
      link override Signal_Limit/_maxval: Value=KOUTP_SetSpd_kph_maxval
      link override Signal_Limit/_minval: Value=KOUTP_SetSpd_kph_minval
      link override Signal_Override/_ovrdflg: Value=KOUTP_SetSpd_kph_ovrdflg
      link override Signal_Override/_ovrdval: Value=KOUTP_SetSpd_kph_ovrdval
  VTQD_ShiftGearPosn_enum_Inproc : FVT_lib/outp/OverrideAndLimit  SystemSampleTime=-1  VariantActivationTime=update diagram  Latency=0  AutoFrameSizeCalculation=off
      link override Signal_Limit/_maxval: Value=KOUTP_ShiftGearPosn_enum_maxval
      link override Signal_Limit/_minval: Value=KOUTP_ShiftGearPosn_enum_minval
      link override Signal_Override/_ovrdflg: Value=KOUTP_ShiftGearPosn_enum_ovrdflg
      link override Signal_Override/_ovrdval: Value=KOUTP_ShiftGearPosn_enum_ovrdval
  VTQD_SpdCtrlMode_enum_Inproc : FVT_lib/outp/OverrideAndLimit  SystemSampleTime=-1  VariantActivationTime=update diagram  Latency=0  AutoFrameSizeCalculation=off
      link override Signal_Limit/_maxval: Value=KOUTP_SpdCtrlMode_enum_maxval
      link override Signal_Limit/_minval: Value=KOUTP_SpdCtrlMode_enum_minval
      link override Signal_Override/_ovrdflg: Value=KOUTP_SpdCtrlMode_enum_ovrdflg
      link override Signal_Override/_ovrdval: Value=KOUTP_SpdCtrlMode_enum_ovrdval
  VTQD_SpdCtrlSta_flg_Inproc : FVT_lib/outp/OverrideAndLimit  SystemSampleTime=-1  VariantActivationTime=update diagram  Latency=0  AutoFrameSizeCalculation=off
      link override Signal_Limit/_maxval: Value=KOUTP_SpdCtrlSta_flg_maxval
      link override Signal_Limit/_minval: Value=KOUTP_SpdCtrlSta_flg_minval
      link override Signal_Override/_ovrdflg: Value=KOUTP_SpdCtrlSta_flg_ovrdflg
      link override Signal_Override/_ovrdval: Value=KOUTP_SpdCtrlSta_flg_ovrdval
  VTQD_TqSourceFr_enum_Inproc : FVT_lib/outp/OverrideAndLimit  SystemSampleTime=-1  VariantActivationTime=update diagram  Latency=0  AutoFrameSizeCalculation=off
      link override Signal_Limit/_maxval: Value=KOUTP_TqSourceFr_enum_maxval
      link override Signal_Limit/_minval: Value=KOUTP_TqSourceFr_enum_minval
      link override Signal_Override/_ovrdflg: Value=KOUTP_TqSourceFr_enum_ovrdflg
      link override Signal_Override/_ovrdval: Value=KOUTP_TqSourceFr_enum_ovrdval
  VTQD_TqSourceRr_enum_Inproc : FVT_lib/outp/OverrideAndLimit  SystemSampleTime=-1  VariantActivationTime=update diagram  Latency=0  AutoFrameSizeCalculation=off
      link override Signal_Limit/_maxval: Value=KOUTP_TqSourceRr_enum_maxval
      link override Signal_Limit/_minval: Value=KOUTP_TqSourceRr_enum_minval
      link override Signal_Override/_ovrdflg: Value=KOUTP_TqSourceRr_enum_ovrdflg
      link override Signal_Override/_ovrdval: Value=KOUTP_TqSourceRr_enum_ovrdval
  VTQR_FrTMTqReq_Nm_Inproc : FVT_lib/outp/OverrideAndLimit  SystemSampleTime=-1  VariantActivationTime=update diagram  Latency=0  AutoFrameSizeCalculation=off
      link override Signal_Limit/_maxval: Value=KOUTP_FrTMTqReq_Nm_maxval
      link override Signal_Limit/_minval: Value=KOUTP_FrTMTqReq_Nm_minval
      link override Signal_Override/_ovrdflg: Value=KOUTP_FrTMTqReq_Nm_ovrdflg
      link override Signal_Override/_ovrdval: Value=KOUTP_FrTMTqReq_Nm_ovrdval
  VTQR_RrTMTqReq_Nm_Inproc : FVT_lib/outp/OverrideAndLimit  SystemSampleTime=-1  VariantActivationTime=update diagram  Latency=0  AutoFrameSizeCalculation=off
      link override Signal_Limit/_maxval: Value=KOUTP_RrTMTqReq_Nm_maxval
      link override Signal_Limit/_minval: Value=KOUTP_RrTMTqReq_Nm_minval
      link override Signal_Override/_ovrdflg: Value=KOUTP_RrTMTqReq_Nm_ovrdflg
      link override Signal_Override/_ovrdval: Value=KOUTP_RrTMTqReq_Nm_ovrdval
  VV2L_ReqOBCV2LEna_enum_Inproc : FVT_lib/outp/OverrideAndLimit  SystemSampleTime=-1  VariantActivationTime=update diagram  Latency=0  AutoFrameSizeCalculation=off
      link override Signal_Limit/_maxval: Value=KOUTP_ReqOBCV2LEna_enum_maxval
      link override Signal_Limit/_minval: Value=KOUTP_ReqOBCV2LEna_enum_minval
      link override Signal_Override/_ovrdflg: Value=KOUTP_ReqOBCV2LEna_enum_ovrdflg
      link override Signal_Override/_ovrdval: Value=KOUTP_ReqOBCV2LEna_enum_ovrdval
  VV2L_ReqV2LIVIPopup_enum_Inproc : FVT_lib/outp/OverrideAndLimit  SystemSampleTime=-1  VariantActivationTime=update diagram  Latency=0  AutoFrameSizeCalculation=off
      link override Signal_Limit/_maxval: Value=KOUTP_ReqV2LIVIPopup_enum_maxval
      link override Signal_Limit/_minval: Value=KOUTP_ReqV2LIVIPopup_enum_minval
      link override Signal_Override/_ovrdflg: Value=KOUTP_ReqV2LIVIPopup_enum_ovrdflg
      link override Signal_Override/_ovrdval: Value=KOUTP_ReqV2LIVIPopup_enum_ovrdval
  VVMC_ACCComfortBandLower_mps2_Inproc : FVT_lib/outp/OverrideAndLimit  SystemSampleTime=-1  VariantActivationTime=update diagram  Latency=0  AutoFrameSizeCalculation=off
      link override Signal_Limit/_maxval: Value=KOUTP_ACCComfortBandLower_mps2_maxval
      link override Signal_Limit/_minval: Value=KOUTP_ACCComfortBandLower_mps2_minval
      link override Signal_Override/_ovrdflg: Value=KOUTP_ACCComfortBandLower_mps2_ovrdflg
      link override Signal_Override/_ovrdval: Value=KOUTP_ACCComfortBandLower_mps2_ovrdval
  VVMC_ACCComfortBandUpper_mps2_Inproc : FVT_lib/outp/OverrideAndLimit  SystemSampleTime=-1  VariantActivationTime=update diagram  Latency=0  AutoFrameSizeCalculation=off
      link override Signal_Limit/_maxval: Value=KOUTP_ACCComfortBandUpper_mps2_maxval
      link override Signal_Limit/_minval: Value=KOUTP_ACCComfortBandUpper_mps2_minval
      link override Signal_Override/_ovrdflg: Value=KOUTP_ACCComfortBandUpper_mps2_ovrdflg
      link override Signal_Override/_ovrdval: Value=KOUTP_ACCComfortBandUpper_mps2_ovrdval
  VVMC_ACCCtrlAvail_flg_Inproc : FVT_lib/outp/OverrideAndLimit  SystemSampleTime=-1  VariantActivationTime=update diagram  Latency=0  AutoFrameSizeCalculation=off
      link override Signal_Limit/_maxval: Value=KOUTP_ACCCtrlAvail_flg_maxval
      link override Signal_Limit/_minval: Value=KOUTP_ACCCtrlAvail_flg_minval
      link override Signal_Override/_ovrdflg: Value=KOUTP_ACCCtrlAvail_flg_ovrdflg
      link override Signal_Override/_ovrdval: Value=KOUTP_ACCCtrlAvail_flg_ovrdval
  VVMC_ACCJerkLowerLimit_mps3_Inproc : FVT_lib/outp/OverrideAndLimit  SystemSampleTime=-1  VariantActivationTime=update diagram  Latency=0  AutoFrameSizeCalculation=off
      link override Signal_Limit/_maxval: Value=KOUTP_ACCJerkLowerLimit_mps3_maxval
      link override Signal_Limit/_minval: Value=KOUTP_ACCJerkLowerLimit_mps3_minval
      link override Signal_Override/_ovrdflg: Value=KOUTP_ACCJerkLowerLimit_mps3_ovrdflg
      link override Signal_Override/_ovrdval: Value=KOUTP_ACCJerkLowerLimit_mps3_ovrdval
  VVMC_ACCJerkUpperLimit_mps3_Inproc : FVT_lib/outp/OverrideAndLimit  SystemSampleTime=-1  VariantActivationTime=update diagram  Latency=0  AutoFrameSizeCalculation=off
      link override Signal_Limit/_maxval: Value=KOUTP_ACCJerkUpperLimit_mps3_maxval
      link override Signal_Limit/_minval: Value=KOUTP_ACCJerkUpperLimit_mps3_minval
      link override Signal_Override/_ovrdflg: Value=KOUTP_ACCJerkUpperLimit_mps3_ovrdflg
      link override Signal_Override/_ovrdval: Value=KOUTP_ACCJerkUpperLimit_mps3_ovrdval
  VVMC_ACCObjDist_m_Inproc : FVT_lib/outp/OverrideAndLimit  SystemSampleTime=-1  VariantActivationTime=update diagram  Latency=0  AutoFrameSizeCalculation=off
      link override Signal_Limit/_maxval: Value=KOUTP_ACCObjDist_m_maxval
      link override Signal_Limit/_minval: Value=KOUTP_ACCObjDist_m_minval
      link override Signal_Override/_ovrdflg: Value=KOUTP_ACCObjDist_m_ovrdflg
      link override Signal_Override/_ovrdval: Value=KOUTP_ACCObjDist_m_ovrdval
  VVMC_ACCObjDstLvl_enum_Inproc : FVT_lib/outp/OverrideAndLimit  SystemSampleTime=-1  VariantActivationTime=update diagram  Latency=0  AutoFrameSizeCalculation=off
      link override Signal_Limit/_maxval: Value=KOUTP_ACCObjDstLvl_enum_maxval
      link override Signal_Limit/_minval: Value=KOUTP_ACCObjDstLvl_enum_minval
      link override Signal_Override/_ovrdflg: Value=KOUTP_ACCObjDstLvl_enum_ovrdflg
      link override Signal_Override/_ovrdval: Value=KOUTP_ACCObjDstLvl_enum_ovrdval
  VVMC_ACCObjRelSpd_mps_Inproc : FVT_lib/outp/OverrideAndLimit  SystemSampleTime=-1  VariantActivationTime=update diagram  Latency=0  AutoFrameSizeCalculation=off
      link override Signal_Limit/_maxval: Value=KOUTP_ACCObjRelSpd_mps_maxval
      link override Signal_Limit/_minval: Value=KOUTP_ACCObjRelSpd_mps_minval
      link override Signal_Override/_ovrdflg: Value=KOUTP_ACCObjRelSpd_mps_ovrdflg
      link override Signal_Override/_ovrdval: Value=KOUTP_ACCObjRelSpd_mps_ovrdval
  VVMC_ACCPedalOvrd_flg_Inproc : FVT_lib/outp/OverrideAndLimit  SystemSampleTime=-1  VariantActivationTime=update diagram  Latency=0  AutoFrameSizeCalculation=off
      link override Signal_Limit/_maxval: Value=KOUTP_ACCPedalOvrd_flg_maxval
      link override Signal_Limit/_minval: Value=KOUTP_ACCPedalOvrd_flg_minval
      link override Signal_Override/_ovrdflg: Value=KOUTP_ACCPedalOvrd_flg_ovrdflg
      link override Signal_Override/_ovrdval: Value=KOUTP_ACCPedalOvrd_flg_ovrdval
  VVMC_ACCRequiredAccel_mps2_Inproc : FVT_lib/outp/OverrideAndLimit  SystemSampleTime=-1  VariantActivationTime=update diagram  Latency=0  AutoFrameSizeCalculation=off
      link override Signal_Limit/_maxval: Value=KOUTP_ACCRequiredAccel_mps2_maxval
      link override Signal_Limit/_minval: Value=KOUTP_ACCRequiredAccel_mps2_minval
      link override Signal_Override/_ovrdflg: Value=KOUTP_ACCRequiredAccel_mps2_ovrdflg
      link override Signal_Override/_ovrdval: Value=KOUTP_ACCRequiredAccel_mps2_ovrdval
  VVMC_ACCTakeoverReq_flg_Inproc : FVT_lib/outp/OverrideAndLimit  SystemSampleTime=-1  VariantActivationTime=update diagram  Latency=0  AutoFrameSizeCalculation=off
      link override Signal_Limit/_maxval: Value=KOUTP_ACCTakeoverReq_flg_maxval
      link override Signal_Limit/_minval: Value=KOUTP_ACCTakeoverReq_flg_minval
      link override Signal_Override/_ovrdflg: Value=KOUTP_ACCTakeoverReq_flg_ovrdflg
      link override Signal_Override/_ovrdval: Value=KOUTP_ACCTakeoverReq_flg_ovrdval
  VVMC_ACCVehHoldReq_flg_Inproc : FVT_lib/outp/OverrideAndLimit  SystemSampleTime=-1  VariantActivationTime=update diagram  Latency=0  AutoFrameSizeCalculation=off
      link override Signal_Limit/_maxval: Value=KOUTP_ACCVehHoldReq_flg_maxval
      link override Signal_Limit/_minval: Value=KOUTP_ACCVehHoldReq_flg_minval
      link override Signal_Override/_ovrdflg: Value=KOUTP_ACCVehHoldReq_flg_ovrdflg
      link override Signal_Override/_ovrdval: Value=KOUTP_ACCVehHoldReq_flg_ovrdval
  VVMC_ADASACCSta_enum_Inproc : FVT_lib/outp/OverrideAndLimit  SystemSampleTime=-1  VariantActivationTime=update diagram  Latency=0  AutoFrameSizeCalculation=off
      link override Signal_Limit/_maxval: Value=KOUTP_ADASACCSta_enum_maxval
      link override Signal_Limit/_minval: Value=KOUTP_ADASACCSta_enum_minval
      link override Signal_Override/_ovrdflg: Value=KOUTP_ADASACCSta_enum_ovrdflg
      link override Signal_Override/_ovrdval: Value=KOUTP_ADASACCSta_enum_ovrdval
  VVMC_ADASAEBReq_enum_Inproc : FVT_lib/outp/OverrideAndLimit  SystemSampleTime=-1  VariantActivationTime=update diagram  Latency=0  AutoFrameSizeCalculation=off
      link override Signal_Limit/_maxval: Value=KOUTP_ADASAEBReq_enum_maxval
      link override Signal_Limit/_minval: Value=KOUTP_ADASAEBReq_enum_minval
      link override Signal_Override/_ovrdflg: Value=KOUTP_ADASAEBReq_enum_ovrdflg
      link override Signal_Override/_ovrdval: Value=KOUTP_ADASAEBReq_enum_ovrdval
  VVMC_ADASAEBSta_enum_Inproc : FVT_lib/outp/OverrideAndLimit  SystemSampleTime=-1  VariantActivationTime=update diagram  Latency=0  AutoFrameSizeCalculation=off
      link override Signal_Limit/_maxval: Value=KOUTP_ADASAEBSta_enum_maxval
      link override Signal_Limit/_minval: Value=KOUTP_ADASAEBSta_enum_minval
      link override Signal_Override/_ovrdflg: Value=KOUTP_ADASAEBSta_enum_ovrdflg
      link override Signal_Override/_ovrdval: Value=KOUTP_ADASAEBSta_enum_ovrdval
  VVMC_ADASCAMSpdLim_enum_Inproc : FVT_lib/outp/OverrideAndLimit  SystemSampleTime=-1  VariantActivationTime=update diagram  Latency=0  AutoFrameSizeCalculation=off
      link override Signal_Limit/_maxval: Value=KOUTP_ADASCAMSpdLim_enum_maxval
      link override Signal_Limit/_minval: Value=KOUTP_ADASCAMSpdLim_enum_minval
      link override Signal_Override/_ovrdflg: Value=KOUTP_ADASCAMSpdLim_enum_ovrdflg
      link override Signal_Override/_ovrdval: Value=KOUTP_ADASCAMSpdLim_enum_ovrdval
  VVMC_ADASDBSReq_enum_Inproc : FVT_lib/outp/OverrideAndLimit  SystemSampleTime=-1  VariantActivationTime=update diagram  Latency=0  AutoFrameSizeCalculation=off
      link override Signal_Limit/_maxval: Value=KOUTP_ADASDBSReq_enum_maxval
      link override Signal_Limit/_minval: Value=KOUTP_ADASDBSReq_enum_minval
      link override Signal_Override/_ovrdflg: Value=KOUTP_ADASDBSReq_enum_ovrdflg
      link override Signal_Override/_ovrdval: Value=KOUTP_ADASDBSReq_enum_ovrdval
  VVMC_ADASFCWMute_flg_Inproc : FVT_lib/outp/OverrideAndLimit  SystemSampleTime=-1  VariantActivationTime=update diagram  Latency=0  AutoFrameSizeCalculation=off
      link override Signal_Limit/_maxval: Value=KOUTP_ADASFCWMute_flg_maxval
      link override Signal_Limit/_minval: Value=KOUTP_ADASFCWMute_flg_minval
      link override Signal_Override/_ovrdflg: Value=KOUTP_ADASFCWMute_flg_ovrdflg
      link override Signal_Override/_ovrdval: Value=KOUTP_ADASFCWMute_flg_ovrdval
  VVMC_ADASFCWSta_enum_Inproc : FVT_lib/outp/OverrideAndLimit  SystemSampleTime=-1  VariantActivationTime=update diagram  Latency=0  AutoFrameSizeCalculation=off
      link override Signal_Limit/_maxval: Value=KOUTP_ADASFCWSta_enum_maxval
      link override Signal_Limit/_minval: Value=KOUTP_ADASFCWSta_enum_minval
      link override Signal_Override/_ovrdflg: Value=KOUTP_ADASFCWSta_enum_ovrdflg
      link override Signal_Override/_ovrdval: Value=KOUTP_ADASFCWSta_enum_ovrdval
  VVMC_ADASFaultSta_flg_Inproc : FVT_lib/outp/OverrideAndLimit  SystemSampleTime=-1  VariantActivationTime=update diagram  Latency=0  AutoFrameSizeCalculation=off
      link override Signal_Limit/_maxval: Value=KOUTP_ADASFaultSta_flg_maxval
      link override Signal_Limit/_minval: Value=KOUTP_ADASFaultSta_flg_minval
      link override Signal_Override/_ovrdflg: Value=KOUTP_ADASFaultSta_flg_ovrdflg
      link override Signal_Override/_ovrdval: Value=KOUTP_ADASFaultSta_flg_ovrdval
  VVMC_ADASFltWrnReq_flg_Inproc : FVT_lib/outp/OverrideAndLimit  SystemSampleTime=-1  VariantActivationTime=update diagram  Latency=0  AutoFrameSizeCalculation=off
      link override Signal_Limit/_maxval: Value=KOUTP_ADASFltWrnReq_flg_maxval
      link override Signal_Limit/_minval: Value=KOUTP_ADASFltWrnReq_flg_minval
      link override Signal_Override/_ovrdflg: Value=KOUTP_ADASFltWrnReq_flg_ovrdflg
      link override Signal_Override/_ovrdval: Value=KOUTP_ADASFltWrnReq_flg_ovrdval
  VVMC_ADASForceIdle_flg_Inproc : FVT_lib/outp/OverrideAndLimit  SystemSampleTime=-1  VariantActivationTime=update diagram  Latency=0  AutoFrameSizeCalculation=off
      link override Signal_Limit/_maxval: Value=KOUTP_ADASForceIdle_flg_maxval
      link override Signal_Limit/_minval: Value=KOUTP_ADASForceIdle_flg_minval
      link override Signal_Override/_ovrdflg: Value=KOUTP_ADASForceIdle_flg_ovrdflg
      link override Signal_Override/_ovrdval: Value=KOUTP_ADASForceIdle_flg_ovrdval
  VVMC_ADASISASta_enum_Inproc : FVT_lib/outp/OverrideAndLimit  SystemSampleTime=-1  VariantActivationTime=update diagram  Latency=0  AutoFrameSizeCalculation=off
      link override Signal_Limit/_maxval: Value=KOUTP_ADASISASta_enum_maxval
      link override Signal_Limit/_minval: Value=KOUTP_ADASISASta_enum_minval
      link override Signal_Override/_ovrdflg: Value=KOUTP_ADASISASta_enum_ovrdflg
      link override Signal_Override/_ovrdval: Value=KOUTP_ADASISASta_enum_ovrdval
  VVMC_ADASLDWMute_flg_Inproc : FVT_lib/outp/OverrideAndLimit  SystemSampleTime=-1  VariantActivationTime=update diagram  Latency=0  AutoFrameSizeCalculation=off
      link override Signal_Limit/_maxval: Value=KOUTP_ADASLDWMute_flg_maxval
      link override Signal_Limit/_minval: Value=KOUTP_ADASLDWMute_flg_minval
      link override Signal_Override/_ovrdflg: Value=KOUTP_ADASLDWMute_flg_ovrdflg
      link override Signal_Override/_ovrdval: Value=KOUTP_ADASLDWMute_flg_ovrdval
  VVMC_ADASLDWSta_enum_Inproc : FVT_lib/outp/OverrideAndLimit  SystemSampleTime=-1  VariantActivationTime=update diagram  Latency=0  AutoFrameSizeCalculation=off
      link override Signal_Limit/_maxval: Value=KOUTP_ADASLDWSta_enum_maxval
      link override Signal_Limit/_minval: Value=KOUTP_ADASLDWSta_enum_minval
      link override Signal_Override/_ovrdflg: Value=KOUTP_ADASLDWSta_enum_ovrdflg
      link override Signal_Override/_ovrdval: Value=KOUTP_ADASLDWSta_enum_ovrdval
  VVMC_ADASLFCHandsOffWarning_enum_Inproc : FVT_lib/outp/OverrideAndLimit  SystemSampleTime=-1  VariantActivationTime=update diagram  Latency=0  AutoFrameSizeCalculation=off
      link override Signal_Limit/_maxval: Value=KOUTP_ADASLFCHandsOffWarning_enum_maxval
      link override Signal_Limit/_minval: Value=KOUTP_ADASLFCHandsOffWarning_enum_minval
      link override Signal_Override/_ovrdflg: Value=KOUTP_ADASLFCHandsOffWarning_enum_ovrdflg
      link override Signal_Override/_ovrdval: Value=KOUTP_ADASLFCHandsOffWarning_enum_ovrdval
  VVMC_ADASLFCSta_enum_Inproc : FVT_lib/outp/OverrideAndLimit  SystemSampleTime=-1  VariantActivationTime=update diagram  Latency=0  AutoFrameSizeCalculation=off
      link override Signal_Limit/_maxval: Value=KOUTP_ADASLFCSta_enum_maxval
      link override Signal_Limit/_minval: Value=KOUTP_ADASLFCSta_enum_minval
      link override Signal_Override/_ovrdflg: Value=KOUTP_ADASLFCSta_enum_ovrdflg
      link override Signal_Override/_ovrdval: Value=KOUTP_ADASLFCSta_enum_ovrdval
  VVMC_ADASLFCWarnSound_enum_Inproc : FVT_lib/outp/OverrideAndLimit  SystemSampleTime=-1  VariantActivationTime=update diagram  Latency=0  AutoFrameSizeCalculation=off
      link override Signal_Limit/_maxval: Value=KOUTP_ADASLFCWarnSound_enum_maxval
      link override Signal_Limit/_minval: Value=KOUTP_ADASLFCWarnSound_enum_minval
      link override Signal_Override/_ovrdflg: Value=KOUTP_ADASLFCWarnSound_enum_ovrdflg
      link override Signal_Override/_ovrdval: Value=KOUTP_ADASLFCWarnSound_enum_ovrdval
  VVMC_ADASLKASta_enum_Inproc : FVT_lib/outp/OverrideAndLimit  SystemSampleTime=-1  VariantActivationTime=update diagram  Latency=0  AutoFrameSizeCalculation=off
      link override Signal_Limit/_maxval: Value=KOUTP_ADASLKASta_enum_maxval
      link override Signal_Limit/_minval: Value=KOUTP_ADASLKASta_enum_minval
      link override Signal_Override/_ovrdflg: Value=KOUTP_ADASLKASta_enum_ovrdflg
      link override Signal_Override/_ovrdval: Value=KOUTP_ADASLKASta_enum_ovrdval
  VVMC_ADASLaneModeL_enum_Inproc : FVT_lib/outp/OverrideAndLimit  SystemSampleTime=-1  VariantActivationTime=update diagram  Latency=0  AutoFrameSizeCalculation=off
      link override Signal_Limit/_maxval: Value=KOUTP_ADASLaneModeL_enum_maxval
      link override Signal_Limit/_minval: Value=KOUTP_ADASLaneModeL_enum_minval
      link override Signal_Override/_ovrdflg: Value=KOUTP_ADASLaneModeL_enum_ovrdflg
      link override Signal_Override/_ovrdval: Value=KOUTP_ADASLaneModeL_enum_ovrdval
  VVMC_ADASLaneModeR_enum_Inproc : FVT_lib/outp/OverrideAndLimit  SystemSampleTime=-1  VariantActivationTime=update diagram  Latency=0  AutoFrameSizeCalculation=off
      link override Signal_Limit/_maxval: Value=KOUTP_ADASLaneModeR_enum_maxval
      link override Signal_Limit/_minval: Value=KOUTP_ADASLaneModeR_enum_minval
      link override Signal_Override/_ovrdflg: Value=KOUTP_ADASLaneModeR_enum_ovrdflg
      link override Signal_Override/_ovrdval: Value=KOUTP_ADASLaneModeR_enum_ovrdval
  VVMC_ADASLanecurveL_raw32_Inproc : FVT_lib/outp/OverrideAndLimit  SystemSampleTime=-1  VariantActivationTime=update diagram  Latency=0  AutoFrameSizeCalculation=off
      link override Signal_Limit/_maxval: Value=KOUTP_ADASLanecurveL_raw32_maxval
      link override Signal_Limit/_minval: Value=KOUTP_ADASLanecurveL_raw32_minval
      link override Signal_Override/_ovrdflg: Value=KOUTP_ADASLanecurveL_raw32_ovrdflg
      link override Signal_Override/_ovrdval: Value=KOUTP_ADASLanecurveL_raw32_ovrdval
  VVMC_ADASLanecurveR_raw32_Inproc : FVT_lib/outp/OverrideAndLimit  SystemSampleTime=-1  VariantActivationTime=update diagram  Latency=0  AutoFrameSizeCalculation=off
      link override Signal_Limit/_maxval: Value=KOUTP_ADASLanecurveR_raw32_maxval
      link override Signal_Limit/_minval: Value=KOUTP_ADASLanecurveR_raw32_minval
      link override Signal_Override/_ovrdflg: Value=KOUTP_ADASLanecurveR_raw32_ovrdflg
      link override Signal_Override/_ovrdval: Value=KOUTP_ADASLanecurveR_raw32_ovrdval
  VVMC_ADASLanetypeL_enum_Inproc : FVT_lib/outp/OverrideAndLimit  SystemSampleTime=-1  VariantActivationTime=update diagram  Latency=0  AutoFrameSizeCalculation=off
      link override Signal_Limit/_maxval: Value=KOUTP_ADASLanetypeL_enum_maxval
      link override Signal_Limit/_minval: Value=KOUTP_ADASLanetypeL_enum_minval
      link override Signal_Override/_ovrdflg: Value=KOUTP_ADASLanetypeL_enum_ovrdflg
      link override Signal_Override/_ovrdval: Value=KOUTP_ADASLanetypeL_enum_ovrdval
  VVMC_ADASLanetypeR_enum_Inproc : FVT_lib/outp/OverrideAndLimit  SystemSampleTime=-1  VariantActivationTime=update diagram  Latency=0  AutoFrameSizeCalculation=off
      link override Signal_Limit/_maxval: Value=KOUTP_ADASLanetypeR_enum_maxval
      link override Signal_Limit/_minval: Value=KOUTP_ADASLanetypeR_enum_minval
      link override Signal_Override/_ovrdflg: Value=KOUTP_ADASLanetypeR_enum_ovrdflg
      link override Signal_Override/_ovrdval: Value=KOUTP_ADASLanetypeR_enum_ovrdval
  VVMC_ADASSLIFSpdLim_enum_Inproc : FVT_lib/outp/OverrideAndLimit  SystemSampleTime=-1  VariantActivationTime=update diagram  Latency=0  AutoFrameSizeCalculation=off
      link override Signal_Limit/_maxval: Value=KOUTP_ADASSLIFSpdLim_enum_maxval
      link override Signal_Limit/_minval: Value=KOUTP_ADASSLIFSpdLim_enum_minval
      link override Signal_Override/_ovrdflg: Value=KOUTP_ADASSLIFSpdLim_enum_ovrdflg
      link override Signal_Override/_ovrdval: Value=KOUTP_ADASSLIFSpdLim_enum_ovrdval
  VVMC_ADASSLIFSta_enum_Inproc : FVT_lib/outp/OverrideAndLimit  SystemSampleTime=-1  VariantActivationTime=update diagram  Latency=0  AutoFrameSizeCalculation=off
      link override Signal_Limit/_maxval: Value=KOUTP_ADASSLIFSta_enum_maxval
      link override Signal_Limit/_minval: Value=KOUTP_ADASSLIFSta_enum_minval
      link override Signal_Override/_ovrdflg: Value=KOUTP_ADASSLIFSta_enum_ovrdflg
      link override Signal_Override/_ovrdval: Value=KOUTP_ADASSLIFSta_enum_ovrdval
  VVMC_ADASShftPosnReqA_flg_Inproc : FVT_lib/outp/OverrideAndLimit  SystemSampleTime=-1  VariantActivationTime=update diagram  Latency=0  AutoFrameSizeCalculation=off
      link override Signal_Limit/_maxval: Value=KOUTP_ADASShftPosnReqA_flg_maxval
      link override Signal_Limit/_minval: Value=KOUTP_ADASShftPosnReqA_flg_minval
      link override Signal_Override/_ovrdflg: Value=KOUTP_ADASShftPosnReqA_flg_ovrdflg
      link override Signal_Override/_ovrdval: Value=KOUTP_ADASShftPosnReqA_flg_ovrdval
  VVMC_ADASShftPosnReq_enum_Inproc : FVT_lib/outp/OverrideAndLimit  SystemSampleTime=-1  VariantActivationTime=update diagram  Latency=0  AutoFrameSizeCalculation=off
      link override Signal_Limit/_maxval: Value=KOUTP_ADASShftPosnReq_enum_maxval
      link override Signal_Limit/_minval: Value=KOUTP_ADASShftPosnReq_enum_minval
      link override Signal_Override/_ovrdflg: Value=KOUTP_ADASShftPosnReq_enum_ovrdflg
      link override Signal_Override/_ovrdval: Value=KOUTP_ADASShftPosnReq_enum_ovrdval
  VVMC_ADASVehSpdLim_raw32_Inproc : FVT_lib/outp/OverrideAndLimit  SystemSampleTime=-1  VariantActivationTime=update diagram  Latency=0  AutoFrameSizeCalculation=off
      link override Signal_Limit/_maxval: Value=KOUTP_ADASVehSpdLim_raw32_maxval
      link override Signal_Limit/_minval: Value=KOUTP_ADASVehSpdLim_raw32_minval
      link override Signal_Override/_ovrdflg: Value=KOUTP_ADASVehSpdLim_raw32_ovrdflg
      link override Signal_Override/_ovrdval: Value=KOUTP_ADASVehSpdLim_raw32_ovrdval
  VVMC_ADASWarningMsg_enum_Inproc : FVT_lib/outp/OverrideAndLimit  SystemSampleTime=-1  VariantActivationTime=update diagram  Latency=0  AutoFrameSizeCalculation=off
      link override Signal_Limit/_maxval: Value=KOUTP_ADASWarningMsg_enum_maxval
      link override Signal_Limit/_minval: Value=KOUTP_ADASWarningMsg_enum_minval
      link override Signal_Override/_ovrdflg: Value=KOUTP_ADASWarningMsg_enum_ovrdflg
      link override Signal_Override/_ovrdval: Value=KOUTP_ADASWarningMsg_enum_ovrdval
  VVMC_AEBVehHoldReq_flg_Inproc : FVT_lib/outp/OverrideAndLimit  SystemSampleTime=-1  VariantActivationTime=update diagram  Latency=0  AutoFrameSizeCalculation=off
      link override Signal_Limit/_maxval: Value=KOUTP_AEBVehHoldReq_flg_maxval
      link override Signal_Limit/_minval: Value=KOUTP_AEBVehHoldReq_flg_minval
      link override Signal_Override/_ovrdflg: Value=KOUTP_AEBVehHoldReq_flg_ovrdflg
      link override Signal_Override/_ovrdval: Value=KOUTP_AEBVehHoldReq_flg_ovrdval
  VVMC_APSCtrlAvail_flg_Inproc : FVT_lib/outp/OverrideAndLimit  SystemSampleTime=-1  VariantActivationTime=update diagram  Latency=0  AutoFrameSizeCalculation=off
      link override Signal_Limit/_maxval: Value=KOUTP_APSCtrlAvail_flg_maxval
      link override Signal_Limit/_minval: Value=KOUTP_APSCtrlAvail_flg_minval
      link override Signal_Override/_ovrdflg: Value=KOUTP_APSCtrlAvail_flg_ovrdflg
      link override Signal_Override/_ovrdval: Value=KOUTP_APSCtrlAvail_flg_ovrdval
  VVMC_APSDecReqA_flg_Inproc : FVT_lib/outp/OverrideAndLimit  SystemSampleTime=-1  VariantActivationTime=update diagram  Latency=0  AutoFrameSizeCalculation=off
      link override Signal_Limit/_maxval: Value=KOUTP_APSDecReqA_flg_maxval
      link override Signal_Limit/_minval: Value=KOUTP_APSDecReqA_flg_minval
      link override Signal_Override/_ovrdflg: Value=KOUTP_APSDecReqA_flg_ovrdflg
      link override Signal_Override/_ovrdval: Value=KOUTP_APSDecReqA_flg_ovrdval
  VVMC_APSDecReq_mps2_Inproc : FVT_lib/outp/OverrideAndLimit  SystemSampleTime=-1  VariantActivationTime=update diagram  Latency=0  AutoFrameSizeCalculation=off
      link override Signal_Limit/_maxval: Value=KOUTP_APSDecReq_mps2_maxval
      link override Signal_Limit/_minval: Value=KOUTP_APSDecReq_mps2_minval
      link override Signal_Override/_ovrdflg: Value=KOUTP_APSDecReq_mps2_ovrdflg
      link override Signal_Override/_ovrdval: Value=KOUTP_APSDecReq_mps2_ovrdval
  VVMC_APSReq_enum_Inproc : FVT_lib/outp/OverrideAndLimit  SystemSampleTime=-1  VariantActivationTime=update diagram  Latency=0  AutoFrameSizeCalculation=off
      link override Signal_Limit/_maxval: Value=KOUTP_APSReq_enum_maxval
      link override Signal_Limit/_minval: Value=KOUTP_APSReq_enum_minval
      link override Signal_Override/_ovrdflg: Value=KOUTP_APSReq_enum_ovrdflg
      link override Signal_Override/_ovrdval: Value=KOUTP_APSReq_enum_ovrdval
  VVMC_APSStaSys_enum_Inproc : FVT_lib/outp/OverrideAndLimit  SystemSampleTime=-1  VariantActivationTime=update diagram  Latency=0  AutoFrameSizeCalculation=off
      link override Signal_Limit/_maxval: Value=KOUTP_APSStaSys_enum_maxval
      link override Signal_Limit/_minval: Value=KOUTP_APSStaSys_enum_minval
      link override Signal_Override/_ovrdflg: Value=KOUTP_APSStaSys_enum_ovrdflg
      link override Signal_Override/_ovrdval: Value=KOUTP_APSStaSys_enum_ovrdval
  VVMC_AccCalcuPID_mps2_Inproc : FVT_lib/outp/OverrideAndLimit  SystemSampleTime=-1  VariantActivationTime=update diagram  Latency=0  AutoFrameSizeCalculation=off
      link override Signal_Limit/_maxval: Value=KOUTP_AccCalcuPID_mps2_maxval
      link override Signal_Limit/_minval: Value=KOUTP_AccCalcuPID_mps2_minval
      link override Signal_Override/_ovrdflg: Value=KOUTP_AccCalcuPID_mps2_ovrdflg
      link override Signal_Override/_ovrdval: Value=KOUTP_AccCalcuPID_mps2_ovrdval
  VVMC_CAASActive_flg_Inproc : FVT_lib/outp/OverrideAndLimit  SystemSampleTime=-1  VariantActivationTime=update diagram  Latency=0  AutoFrameSizeCalculation=off
      link override Signal_Limit/_maxval: Value=KOUTP_CAASActive_flg_maxval
      link override Signal_Limit/_minval: Value=KOUTP_CAASActive_flg_minval
      link override Signal_Override/_ovrdflg: Value=KOUTP_CAASActive_flg_ovrdflg
      link override Signal_Override/_ovrdval: Value=KOUTP_CAASActive_flg_ovrdval
  VVMC_CAASCtrlAvail_flg_Inproc : FVT_lib/outp/OverrideAndLimit  SystemSampleTime=-1  VariantActivationTime=update diagram  Latency=0  AutoFrameSizeCalculation=off
      link override Signal_Limit/_maxval: Value=KOUTP_CAASCtrlAvail_flg_maxval
      link override Signal_Limit/_minval: Value=KOUTP_CAASCtrlAvail_flg_minval
      link override Signal_Override/_ovrdflg: Value=KOUTP_CAASCtrlAvail_flg_ovrdflg
      link override Signal_Override/_ovrdval: Value=KOUTP_CAASCtrlAvail_flg_ovrdval
  VVMC_CCCtrlSta_enum_Inproc : FVT_lib/outp/OverrideAndLimit  SystemSampleTime=-1  VariantActivationTime=update diagram  Latency=0  AutoFrameSizeCalculation=off
      link override Signal_Limit/_maxval: Value=KOUTP_CCCtrlSta_enum_maxval
      link override Signal_Limit/_minval: Value=KOUTP_CCCtrlSta_enum_minval
      link override Signal_Override/_ovrdflg: Value=KOUTP_CCCtrlSta_enum_ovrdflg
      link override Signal_Override/_ovrdval: Value=KOUTP_CCCtrlSta_enum_ovrdval
  VVMC_CCMSASpdWar_flg_Inproc : FVT_lib/outp/OverrideAndLimit  SystemSampleTime=-1  VariantActivationTime=update diagram  Latency=0  AutoFrameSizeCalculation=off
      link override Signal_Limit/_maxval: Value=KOUTP_CCMSASpdWar_flg_maxval
      link override Signal_Limit/_minval: Value=KOUTP_CCMSASpdWar_flg_minval
      link override Signal_Override/_ovrdflg: Value=KOUTP_CCMSASpdWar_flg_ovrdflg
      link override Signal_Override/_ovrdval: Value=KOUTP_CCMSASpdWar_flg_ovrdval
  VVMC_DISCReqAcc_mps2_Inproc : FVT_lib/outp/OverrideAndLimit  SystemSampleTime=-1  VariantActivationTime=update diagram  Latency=0  AutoFrameSizeCalculation=off
      link override Signal_Limit/_maxval: Value=KOUTP_DISCReqAcc_mps2_maxval
      link override Signal_Limit/_minval: Value=KOUTP_DISCReqAcc_mps2_minval
      link override Signal_Override/_ovrdflg: Value=KOUTP_DISCReqAcc_mps2_ovrdflg
      link override Signal_Override/_ovrdval: Value=KOUTP_DISCReqAcc_mps2_ovrdval
  VVMC_FCMACCmode_enum_Inproc : FVT_lib/outp/OverrideAndLimit  SystemSampleTime=-1  VariantActivationTime=update diagram  Latency=0  AutoFrameSizeCalculation=off
      link override Signal_Limit/_maxval: Value=KOUTP_FCMACCmode_enum_maxval
      link override Signal_Limit/_minval: Value=KOUTP_FCMACCmode_enum_minval
      link override Signal_Override/_ovrdflg: Value=KOUTP_FCMACCmode_enum_ovrdflg
      link override Signal_Override/_ovrdval: Value=KOUTP_FCMACCmode_enum_ovrdval
  VVMC_FCMLDWFault_flg_Inproc : FVT_lib/outp/OverrideAndLimit  SystemSampleTime=-1  VariantActivationTime=update diagram  Latency=0  AutoFrameSizeCalculation=off
      link override Signal_Limit/_maxval: Value=KOUTP_FCMLDWFault_flg_maxval
      link override Signal_Limit/_minval: Value=KOUTP_FCMLDWFault_flg_minval
      link override Signal_Override/_ovrdflg: Value=KOUTP_FCMLDWFault_flg_ovrdflg
      link override Signal_Override/_ovrdval: Value=KOUTP_FCMLDWFault_flg_ovrdval
  VVMC_FCMLDWRequest_enum_Inproc : FVT_lib/outp/OverrideAndLimit  SystemSampleTime=-1  VariantActivationTime=update diagram  Latency=0  AutoFrameSizeCalculation=off
      link override Signal_Limit/_maxval: Value=KOUTP_FCMLDWRequest_enum_maxval
      link override Signal_Limit/_minval: Value=KOUTP_FCMLDWRequest_enum_minval
      link override Signal_Override/_ovrdflg: Value=KOUTP_FCMLDWRequest_enum_ovrdflg
      link override Signal_Override/_ovrdval: Value=KOUTP_FCMLDWRequest_enum_ovrdval
  VVMC_FeatArbitrFinal_enum_Inproc : FVT_lib/outp/OverrideAndLimit  SystemSampleTime=-1  VariantActivationTime=update diagram  Latency=0  AutoFrameSizeCalculation=off
      link override Signal_Limit/_maxval: Value=KOUTP_FeatArbitrFinal_enum_maxval
      link override Signal_Limit/_minval: Value=KOUTP_FeatArbitrFinal_enum_minval
      link override Signal_Override/_ovrdflg: Value=KOUTP_FeatArbitrFinal_enum_ovrdflg
      link override Signal_Override/_ovrdval: Value=KOUTP_FeatArbitrFinal_enum_ovrdval
  VVMC_FeatArbitrSta_enum_Inproc : FVT_lib/outp/OverrideAndLimit  SystemSampleTime=-1  VariantActivationTime=update diagram  Latency=0  AutoFrameSizeCalculation=off
      link override Signal_Limit/_maxval: Value=KOUTP_FeatArbitrSta_enum_maxval
      link override Signal_Limit/_minval: Value=KOUTP_FeatArbitrSta_enum_minval
      link override Signal_Override/_ovrdflg: Value=KOUTP_FeatArbitrSta_enum_ovrdflg
      link override Signal_Override/_ovrdval: Value=KOUTP_FeatArbitrSta_enum_ovrdval
  VVMC_FeatReqSpd_kph_Inproc : FVT_lib/outp/OverrideAndLimit  SystemSampleTime=-1  VariantActivationTime=update diagram  Latency=0  AutoFrameSizeCalculation=off
      link override Signal_Limit/_maxval: Value=KOUTP_FeatReqSpd_kph_maxval
      link override Signal_Limit/_minval: Value=KOUTP_FeatReqSpd_kph_minval
      link override Signal_Override/_ovrdflg: Value=KOUTP_FeatReqSpd_kph_ovrdflg
      link override Signal_Override/_ovrdval: Value=KOUTP_FeatReqSpd_kph_ovrdval
  VVMC_FeatSetSpdFinal_raw32_Inproc : FVT_lib/outp/OverrideAndLimit  SystemSampleTime=-1  VariantActivationTime=update diagram  Latency=0  AutoFrameSizeCalculation=off
      link override Signal_Limit/_maxval: Value=KOUTP_FeatSetSpdFinal_raw32_maxval
      link override Signal_Limit/_minval: Value=KOUTP_FeatSetSpdFinal_raw32_minval
      link override Signal_Override/_ovrdflg: Value=KOUTP_FeatSetSpdFinal_raw32_ovrdflg
      link override Signal_Override/_ovrdval: Value=KOUTP_FeatSetSpdFinal_raw32_ovrdval
  VVMC_ForceLowBeam_enum_Inproc : FVT_lib/outp/OverrideAndLimit  SystemSampleTime=-1  VariantActivationTime=update diagram  Latency=0  AutoFrameSizeCalculation=off
      link override Signal_Limit/_maxval: Value=KOUTP_ForceLowBeam_enum_maxval
      link override Signal_Limit/_minval: Value=KOUTP_ForceLowBeam_enum_minval
      link override Signal_Override/_ovrdflg: Value=KOUTP_ForceLowBeam_enum_ovrdflg
      link override Signal_Override/_ovrdval: Value=KOUTP_ForceLowBeam_enum_ovrdval
  VVMC_FrontRearSlipRatioCtrl_flg_Inproc : FVT_lib/outp/OverrideAndLimit  SystemSampleTime=-1  VariantActivationTime=update diagram  Latency=0  AutoFrameSizeCalculation=off
      link override Signal_Limit/_maxval: Value=KOUTP_FrontRearSlipRatioCtrl_flg_maxval
      link override Signal_Limit/_minval: Value=KOUTP_FrontRearSlipRatioCtrl_flg_minval
      link override Signal_Override/_ovrdflg: Value=KOUTP_FrontRearSlipRatioCtrl_flg_ovrdflg
      link override Signal_Override/_ovrdval: Value=KOUTP_FrontRearSlipRatioCtrl_flg_ovrdval
  VVMC_HazardWarningReq_flg_Inproc : FVT_lib/outp/OverrideAndLimit  SystemSampleTime=-1  VariantActivationTime=update diagram  Latency=0  AutoFrameSizeCalculation=off
      link override Signal_Limit/_maxval: Value=KOUTP_HazardWarningReq_flg_maxval
      link override Signal_Limit/_minval: Value=KOUTP_HazardWarningReq_flg_minval
      link override Signal_Override/_ovrdflg: Value=KOUTP_HazardWarningReq_flg_ovrdflg
      link override Signal_Override/_ovrdval: Value=KOUTP_HazardWarningReq_flg_ovrdval
  VVMC_IMUEnaCmd_flg_Inproc : FVT_lib/outp/OverrideAndLimit  SystemSampleTime=-1  VariantActivationTime=update diagram  Latency=0  AutoFrameSizeCalculation=off
      link override Signal_Limit/_maxval: Value=KOUTP_IMUEnaCmd_flg_maxval
      link override Signal_Limit/_minval: Value=KOUTP_IMUEnaCmd_flg_minval
      link override Signal_Override/_ovrdflg: Value=KOUTP_IMUEnaCmd_flg_ovrdflg
      link override Signal_Override/_ovrdval: Value=KOUTP_IMUEnaCmd_flg_ovrdval
  VVMC_ISOAccLimit_mps2_Inproc : FVT_lib/outp/OverrideAndLimit  SystemSampleTime=-1  VariantActivationTime=update diagram  Latency=0  AutoFrameSizeCalculation=off
      link override Signal_Limit/_maxval: Value=KOUTP_ISOAccLimit_mps2_maxval
      link override Signal_Limit/_minval: Value=KOUTP_ISOAccLimit_mps2_minval
      link override Signal_Override/_ovrdflg: Value=KOUTP_ISOAccLimit_mps2_ovrdflg
      link override Signal_Override/_ovrdval: Value=KOUTP_ISOAccLimit_mps2_ovrdval
  VVMC_ISODecLimit_mps2_Inproc : FVT_lib/outp/OverrideAndLimit  SystemSampleTime=-1  VariantActivationTime=update diagram  Latency=0  AutoFrameSizeCalculation=off
      link override Signal_Limit/_maxval: Value=KOUTP_ISODecLimit_mps2_maxval
      link override Signal_Limit/_minval: Value=KOUTP_ISODecLimit_mps2_minval
      link override Signal_Override/_ovrdflg: Value=KOUTP_ISODecLimit_mps2_ovrdflg
      link override Signal_Override/_ovrdval: Value=KOUTP_ISODecLimit_mps2_ovrdval
  VVMC_ISOJerkLimit_mps3_Inproc : FVT_lib/outp/OverrideAndLimit  SystemSampleTime=-1  VariantActivationTime=update diagram  Latency=0  AutoFrameSizeCalculation=off
      link override Signal_Limit/_maxval: Value=KOUTP_ISOJerkLimit_mps3_maxval
      link override Signal_Limit/_minval: Value=KOUTP_ISOJerkLimit_mps3_minval
      link override Signal_Override/_ovrdflg: Value=KOUTP_ISOJerkLimit_mps3_ovrdflg
      link override Signal_Override/_ovrdval: Value=KOUTP_ISOJerkLimit_mps3_ovrdval
  VVMC_JerkPCT_pct_Inproc : FVT_lib/outp/OverrideAndLimit  SystemSampleTime=-1  VariantActivationTime=update diagram  Latency=0  AutoFrameSizeCalculation=off
      link override Signal_Limit/_maxval: Value=KOUTP_JerkPCT_pct_maxval
      link override Signal_Limit/_minval: Value=KOUTP_JerkPCT_pct_minval
      link override Signal_Override/_ovrdflg: Value=KOUTP_JerkPCT_pct_ovrdflg
      link override Signal_Override/_ovrdval: Value=KOUTP_JerkPCT_pct_ovrdval
  VVMC_LKAHODDisplayWarning_flg_Inproc : FVT_lib/outp/OverrideAndLimit  SystemSampleTime=-1  VariantActivationTime=update diagram  Latency=0  AutoFrameSizeCalculation=off
      link override Signal_Limit/_maxval: Value=KOUTP_LKAHODDisplayWarning_flg_maxval
      link override Signal_Limit/_minval: Value=KOUTP_LKAHODDisplayWarning_flg_minval
      link override Signal_Override/_ovrdflg: Value=KOUTP_LKAHODDisplayWarning_flg_ovrdflg
      link override Signal_Override/_ovrdval: Value=KOUTP_LKAHODDisplayWarning_flg_ovrdval
  VVMC_LKAHODSoundWarning_flg_Inproc : FVT_lib/outp/OverrideAndLimit  SystemSampleTime=-1  VariantActivationTime=update diagram  Latency=0  AutoFrameSizeCalculation=off
      link override Signal_Limit/_maxval: Value=KOUTP_LKAHODSoundWarning_flg_maxval
      link override Signal_Limit/_minval: Value=KOUTP_LKAHODSoundWarning_flg_minval
      link override Signal_Override/_ovrdflg: Value=KOUTP_LKAHODSoundWarning_flg_ovrdflg
      link override Signal_Override/_ovrdval: Value=KOUTP_LKAHODSoundWarning_flg_ovrdval
  VVMC_LKAStrToqReq_Nm_Inproc : FVT_lib/outp/OverrideAndLimit  SystemSampleTime=-1  VariantActivationTime=update diagram  Latency=0  AutoFrameSizeCalculation=off
      link override Signal_Limit/_maxval: Value=KOUTP_LKAStrToqReq_Nm_maxval
      link override Signal_Limit/_minval: Value=KOUTP_LKAStrToqReq_Nm_minval
      link override Signal_Override/_ovrdflg: Value=KOUTP_LKAStrToqReq_Nm_ovrdflg
      link override Signal_Override/_ovrdval: Value=KOUTP_LKAStrToqReq_Nm_ovrdval
  VVMC_LKATOIAct_enum_Inproc : FVT_lib/outp/OverrideAndLimit  SystemSampleTime=-1  VariantActivationTime=update diagram  Latency=0  AutoFrameSizeCalculation=off
      link override Signal_Limit/_maxval: Value=KOUTP_LKATOIAct_enum_maxval
      link override Signal_Limit/_minval: Value=KOUTP_LKATOIAct_enum_minval
      link override Signal_Override/_ovrdflg: Value=KOUTP_LKATOIAct_enum_ovrdflg
      link override Signal_Override/_ovrdval: Value=KOUTP_LKATOIAct_enum_ovrdval
  VVMC_LKATOIFault_flg_Inproc : FVT_lib/outp/OverrideAndLimit  SystemSampleTime=-1  VariantActivationTime=update diagram  Latency=0  AutoFrameSizeCalculation=off
      link override Signal_Limit/_maxval: Value=KOUTP_LKATOIFault_flg_maxval
      link override Signal_Limit/_minval: Value=KOUTP_LKATOIFault_flg_minval
      link override Signal_Override/_ovrdflg: Value=KOUTP_LKATOIFault_flg_ovrdflg
      link override Signal_Override/_ovrdval: Value=KOUTP_LKATOIFault_flg_ovrdval
  VVMC_LVDAACCStatusInformation_flg_Inproc : FVT_lib/outp/OverrideAndLimit  SystemSampleTime=-1  VariantActivationTime=update diagram  Latency=0  AutoFrameSizeCalculation=off
      link override Signal_Limit/_maxval: Value=KOUTP_LVDAACCStatusInformation_flg_maxval
      link override Signal_Limit/_minval: Value=KOUTP_LVDAACCStatusInformation_flg_minval
      link override Signal_Override/_ovrdflg: Value=KOUTP_LVDAACCStatusInformation_flg_ovrdflg
      link override Signal_Override/_ovrdval: Value=KOUTP_LVDAACCStatusInformation_flg_ovrdval
  VVMC_LVDADisabled_flg_Inproc : FVT_lib/outp/OverrideAndLimit  SystemSampleTime=-1  VariantActivationTime=update diagram  Latency=0  AutoFrameSizeCalculation=off
      link override Signal_Limit/_maxval: Value=KOUTP_LVDADisabled_flg_maxval
      link override Signal_Limit/_minval: Value=KOUTP_LVDADisabled_flg_minval
      link override Signal_Override/_ovrdflg: Value=KOUTP_LVDADisabled_flg_ovrdflg
      link override Signal_Override/_ovrdval: Value=KOUTP_LVDADisabled_flg_ovrdval
  VVMC_LVDAFailinfo_flg_Inproc : FVT_lib/outp/OverrideAndLimit  SystemSampleTime=-1  VariantActivationTime=update diagram  Latency=0  AutoFrameSizeCalculation=off
      link override Signal_Limit/_maxval: Value=KOUTP_LVDAFailinfo_flg_maxval
      link override Signal_Limit/_minval: Value=KOUTP_LVDAFailinfo_flg_minval
      link override Signal_Override/_ovrdflg: Value=KOUTP_LVDAFailinfo_flg_ovrdflg
      link override Signal_Override/_ovrdval: Value=KOUTP_LVDAFailinfo_flg_ovrdval
  VVMC_LVDAMuteSta_enum_Inproc : FVT_lib/outp/OverrideAndLimit  SystemSampleTime=-1  VariantActivationTime=update diagram  Latency=0  AutoFrameSizeCalculation=off
      link override Signal_Limit/_maxval: Value=KOUTP_LVDAMuteSta_enum_maxval
      link override Signal_Limit/_minval: Value=KOUTP_LVDAMuteSta_enum_minval
      link override Signal_Override/_ovrdflg: Value=KOUTP_LVDAMuteSta_enum_ovrdflg
      link override Signal_Override/_ovrdval: Value=KOUTP_LVDAMuteSta_enum_ovrdval
  VVMC_LVDAWarning_flg_Inproc : FVT_lib/outp/OverrideAndLimit  SystemSampleTime=-1  VariantActivationTime=update diagram  Latency=0  AutoFrameSizeCalculation=off
      link override Signal_Limit/_maxval: Value=KOUTP_LVDAWarning_flg_maxval
      link override Signal_Limit/_minval: Value=KOUTP_LVDAWarning_flg_minval
      link override Signal_Override/_ovrdflg: Value=KOUTP_LVDAWarning_flg_ovrdflg
      link override Signal_Override/_ovrdval: Value=KOUTP_LVDAWarning_flg_ovrdval
  VVMC_LatAccCtrl_flg_Inproc : FVT_lib/outp/OverrideAndLimit  SystemSampleTime=-1  VariantActivationTime=update diagram  Latency=0  AutoFrameSizeCalculation=off
      link override Signal_Limit/_maxval: Value=KOUTP_LatAccCtrl_flg_maxval
      link override Signal_Limit/_minval: Value=KOUTP_LatAccCtrl_flg_minval
      link override Signal_Override/_ovrdflg: Value=KOUTP_LatAccCtrl_flg_ovrdflg
      link override Signal_Override/_ovrdval: Value=KOUTP_LatAccCtrl_flg_ovrdval
  VVMC_LateralCtrl_flg_Inproc : FVT_lib/outp/OverrideAndLimit  SystemSampleTime=-1  VariantActivationTime=update diagram  Latency=0  AutoFrameSizeCalculation=off
      link override Signal_Limit/_maxval: Value=KOUTP_LateralCtrl_flg_maxval
      link override Signal_Limit/_minval: Value=KOUTP_LateralCtrl_flg_minval
      link override Signal_Override/_ovrdflg: Value=KOUTP_LateralCtrl_flg_ovrdflg
      link override Signal_Override/_ovrdval: Value=KOUTP_LateralCtrl_flg_ovrdval
  VVMC_LeftTurnLightReq_flg_Inproc : FVT_lib/outp/OverrideAndLimit  SystemSampleTime=-1  VariantActivationTime=update diagram  Latency=0  AutoFrameSizeCalculation=off
      link override Signal_Limit/_maxval: Value=KOUTP_LeftTurnLightReq_flg_maxval
      link override Signal_Limit/_minval: Value=KOUTP_LeftTurnLightReq_flg_minval
      link override Signal_Override/_ovrdflg: Value=KOUTP_LeftTurnLightReq_flg_ovrdflg
      link override Signal_Override/_ovrdval: Value=KOUTP_LeftTurnLightReq_flg_ovrdval
  VVMC_LimitPCT_pct_Inproc : FVT_lib/outp/OverrideAndLimit  SystemSampleTime=-1  VariantActivationTime=update diagram  Latency=0  AutoFrameSizeCalculation=off
      link override Signal_Limit/_maxval: Value=KOUTP_LimitPCT_pct_maxval
      link override Signal_Limit/_minval: Value=KOUTP_LimitPCT_pct_minval
      link override Signal_Override/_ovrdflg: Value=KOUTP_LimitPCT_pct_ovrdflg
      link override Signal_Override/_ovrdval: Value=KOUTP_LimitPCT_pct_ovrdval
  VVMC_MSACtrlSta_enum_Inproc : FVT_lib/outp/OverrideAndLimit  SystemSampleTime=-1  VariantActivationTime=update diagram  Latency=0  AutoFrameSizeCalculation=off
      link override Signal_Limit/_maxval: Value=KOUTP_MSACtrlSta_enum_maxval
      link override Signal_Limit/_minval: Value=KOUTP_MSACtrlSta_enum_minval
      link override Signal_Override/_ovrdflg: Value=KOUTP_MSACtrlSta_enum_ovrdflg
      link override Signal_Override/_ovrdval: Value=KOUTP_MSACtrlSta_enum_ovrdval
  VVMC_MeterIndSpeed_raw32_Inproc : FVT_lib/outp/OverrideAndLimit  SystemSampleTime=-1  VariantActivationTime=update diagram  Latency=0  AutoFrameSizeCalculation=off
      link override Signal_Limit/_maxval: Value=KOUTP_MeterIndSpeed_raw32_maxval
      link override Signal_Limit/_minval: Value=KOUTP_MeterIndSpeed_raw32_minval
      link override Signal_Override/_ovrdflg: Value=KOUTP_MeterIndSpeed_raw32_ovrdflg
      link override Signal_Override/_ovrdval: Value=KOUTP_MeterIndSpeed_raw32_ovrdval
  VVMC_RearWhlSlipRatioCtrl_flg_Inproc : FVT_lib/outp/OverrideAndLimit  SystemSampleTime=-1  VariantActivationTime=update diagram  Latency=0  AutoFrameSizeCalculation=off
      link override Signal_Limit/_maxval: Value=KOUTP_RearWhlSlipRatioCtrl_flg_maxval
      link override Signal_Limit/_minval: Value=KOUTP_RearWhlSlipRatioCtrl_flg_minval
      link override Signal_Override/_ovrdflg: Value=KOUTP_RearWhlSlipRatioCtrl_flg_ovrdflg
      link override Signal_Override/_ovrdval: Value=KOUTP_RearWhlSlipRatioCtrl_flg_ovrdval
  VVMC_RightTurnLightReq_flg_Inproc : FVT_lib/outp/OverrideAndLimit  SystemSampleTime=-1  VariantActivationTime=update diagram  Latency=0  AutoFrameSizeCalculation=off
      link override Signal_Limit/_maxval: Value=KOUTP_RightTurnLightReq_flg_maxval
      link override Signal_Limit/_minval: Value=KOUTP_RightTurnLightReq_flg_minval
      link override Signal_Override/_ovrdflg: Value=KOUTP_RightTurnLightReq_flg_ovrdflg
      link override Signal_Override/_ovrdval: Value=KOUTP_RightTurnLightReq_flg_ovrdval
  VVMC_SPD2ACCAct_flg_Inproc : FVT_lib/outp/OverrideAndLimit  SystemSampleTime=-1  VariantActivationTime=update diagram  Latency=0  AutoFrameSizeCalculation=off
      link override Signal_Limit/_maxval: Value=KOUTP_SPD2ACCAct_flg_maxval
      link override Signal_Limit/_minval: Value=KOUTP_SPD2ACCAct_flg_minval
      link override Signal_Override/_ovrdflg: Value=KOUTP_SPD2ACCAct_flg_ovrdflg
      link override Signal_Override/_ovrdval: Value=KOUTP_SPD2ACCAct_flg_ovrdval
  VVMC_SafetyCtrl_flg_Inproc : FVT_lib/outp/OverrideAndLimit  SystemSampleTime=-1  VariantActivationTime=update diagram  Latency=0  AutoFrameSizeCalculation=off
      link override Signal_Limit/_maxval: Value=KOUTP_SafetyCtrl_flg_maxval
      link override Signal_Limit/_minval: Value=KOUTP_SafetyCtrl_flg_minval
      link override Signal_Override/_ovrdflg: Value=KOUTP_SafetyCtrl_flg_ovrdflg
      link override Signal_Override/_ovrdval: Value=KOUTP_SafetyCtrl_flg_ovrdval
  VVMC_SingleWhlSlipRatioCtrl_flg_Inproc : FVT_lib/outp/OverrideAndLimit  SystemSampleTime=-1  VariantActivationTime=update diagram  Latency=0  AutoFrameSizeCalculation=off
      link override Signal_Limit/_maxval: Value=KOUTP_SingleWhlSlipRatioCtrl_flg_maxval
      link override Signal_Limit/_minval: Value=KOUTP_SingleWhlSlipRatioCtrl_flg_minval
      link override Signal_Override/_ovrdflg: Value=KOUTP_SingleWhlSlipRatioCtrl_flg_ovrdflg
      link override Signal_Override/_ovrdval: Value=KOUTP_SingleWhlSlipRatioCtrl_flg_ovrdval
  VVMC_TargetType_enum_Inproc : FVT_lib/outp/OverrideAndLimit  SystemSampleTime=-1  VariantActivationTime=update diagram  Latency=0  AutoFrameSizeCalculation=off
      link override Signal_Limit/_maxval: Value=KOUTP_TargetType_enum_maxval
      link override Signal_Limit/_minval: Value=KOUTP_TargetType_enum_minval
      link override Signal_Override/_ovrdflg: Value=KOUTP_TargetType_enum_ovrdflg
      link override Signal_Override/_ovrdval: Value=KOUTP_TargetType_enum_ovrdval
  VVMC_TimeGapCalcu_s_Inproc : FVT_lib/outp/OverrideAndLimit  SystemSampleTime=-1  VariantActivationTime=update diagram  Latency=0  AutoFrameSizeCalculation=off
      link override Signal_Limit/_maxval: Value=KOUTP_TimeGapCalcu_s_maxval
      link override Signal_Limit/_minval: Value=KOUTP_TimeGapCalcu_s_minval
      link override Signal_Override/_ovrdflg: Value=KOUTP_TimeGapCalcu_s_ovrdflg
      link override Signal_Override/_ovrdval: Value=KOUTP_TimeGapCalcu_s_ovrdval
  VVMC_TimeGapLevel_enum_Inproc : FVT_lib/outp/OverrideAndLimit  SystemSampleTime=-1  VariantActivationTime=update diagram  Latency=0  AutoFrameSizeCalculation=off
      link override Signal_Limit/_maxval: Value=KOUTP_TimeGapLevel_enum_maxval
      link override Signal_Limit/_minval: Value=KOUTP_TimeGapLevel_enum_minval
      link override Signal_Override/_ovrdflg: Value=KOUTP_TimeGapLevel_enum_ovrdflg
      link override Signal_Override/_ovrdval: Value=KOUTP_TimeGapLevel_enum_ovrdval
  VVMC_VMCACCCtrlAvail_flg_Inproc : FVT_lib/outp/OverrideAndLimit  SystemSampleTime=-1  VariantActivationTime=update diagram  Latency=0  AutoFrameSizeCalculation=off
      link override Signal_Limit/_maxval: Value=KOUTP_VMCACCCtrlAvail_flg_maxval
      link override Signal_Limit/_minval: Value=KOUTP_VMCACCCtrlAvail_flg_minval
      link override Signal_Override/_ovrdflg: Value=KOUTP_VMCACCCtrlAvail_flg_ovrdflg
      link override Signal_Override/_ovrdval: Value=KOUTP_VMCACCCtrlAvail_flg_ovrdval
  VVMC_VMCAEBCtrlAvail_flg_Inproc : FVT_lib/outp/OverrideAndLimit  SystemSampleTime=-1  VariantActivationTime=update diagram  Latency=0  AutoFrameSizeCalculation=off
      link override Signal_Limit/_maxval: Value=KOUTP_VMCAEBCtrlAvail_flg_maxval
      link override Signal_Limit/_minval: Value=KOUTP_VMCAEBCtrlAvail_flg_minval
      link override Signal_Override/_ovrdflg: Value=KOUTP_VMCAEBCtrlAvail_flg_ovrdflg
      link override Signal_Override/_ovrdval: Value=KOUTP_VMCAEBCtrlAvail_flg_ovrdval
  VVMC_VMCCCCtrlAvail_flg_Inproc : FVT_lib/outp/OverrideAndLimit  SystemSampleTime=-1  VariantActivationTime=update diagram  Latency=0  AutoFrameSizeCalculation=off
      link override Signal_Limit/_maxval: Value=KOUTP_VMCCCCtrlAvail_flg_maxval
      link override Signal_Limit/_minval: Value=KOUTP_VMCCCCtrlAvail_flg_minval
      link override Signal_Override/_ovrdflg: Value=KOUTP_VMCCCCtrlAvail_flg_ovrdflg
      link override Signal_Override/_ovrdval: Value=KOUTP_VMCCCCtrlAvail_flg_ovrdval
  VVMC_VMCMSACtrlAvail_flg_Inproc : FVT_lib/outp/OverrideAndLimit  SystemSampleTime=-1  VariantActivationTime=update diagram  Latency=0  AutoFrameSizeCalculation=off
      link override Signal_Limit/_maxval: Value=KOUTP_VMCMSACtrlAvail_flg_maxval
      link override Signal_Limit/_minval: Value=KOUTP_VMCMSACtrlAvail_flg_minval
      link override Signal_Override/_ovrdflg: Value=KOUTP_VMCMSACtrlAvail_flg_ovrdflg
      link override Signal_Override/_ovrdval: Value=KOUTP_VMCMSACtrlAvail_flg_ovrdval
  VVMC_VMCRWSActvSta_enum_Inproc : FVT_lib/outp/OverrideAndLimit  SystemSampleTime=-1  VariantActivationTime=update diagram  Latency=0  AutoFrameSizeCalculation=off
      link override Signal_Limit/_maxval: Value=KOUTP_VMCRWSActvSta_enum_maxval
      link override Signal_Limit/_minval: Value=KOUTP_VMCRWSActvSta_enum_minval
      link override Signal_Override/_ovrdflg: Value=KOUTP_VMCRWSActvSta_enum_ovrdflg
      link override Signal_Override/_ovrdval: Value=KOUTP_VMCRWSActvSta_enum_ovrdval
  VVMC_VMCRWSDfctvSta_enum_Inproc : FVT_lib/outp/OverrideAndLimit  SystemSampleTime=-1  VariantActivationTime=update diagram  Latency=0  AutoFrameSizeCalculation=off
      link override Signal_Limit/_maxval: Value=KOUTP_VMCRWSDfctvSta_enum_maxval
      link override Signal_Limit/_minval: Value=KOUTP_VMCRWSDfctvSta_enum_minval
      link override Signal_Override/_ovrdflg: Value=KOUTP_VMCRWSDfctvSta_enum_ovrdflg
      link override Signal_Override/_ovrdval: Value=KOUTP_VMCRWSDfctvSta_enum_ovrdval
  VVMC_VMCRWSPositionReq_mm_Inproc : FVT_lib/outp/OverrideAndLimit  SystemSampleTime=-1  VariantActivationTime=update diagram  Latency=0  AutoFrameSizeCalculation=off
      link override Signal_Limit/_maxval: Value=KOUTP_VMCRWSPositionReq_mm_maxval
      link override Signal_Limit/_minval: Value=KOUTP_VMCRWSPositionReq_mm_minval
      link override Signal_Override/_ovrdflg: Value=KOUTP_VMCRWSPositionReq_mm_ovrdflg
      link override Signal_Override/_ovrdval: Value=KOUTP_VMCRWSPositionReq_mm_ovrdval
  VVMC_VMCSteerFaultRequest_enum_Inproc : FVT_lib/outp/OverrideAndLimit  SystemSampleTime=-1  VariantActivationTime=update diagram  Latency=0  AutoFrameSizeCalculation=off
      link override Signal_Limit/_maxval: Value=KOUTP_VMCSteerFaultRequest_enum_maxval
      link override Signal_Limit/_minval: Value=KOUTP_VMCSteerFaultRequest_enum_minval
      link override Signal_Override/_ovrdflg: Value=KOUTP_VMCSteerFaultRequest_enum_ovrdflg
      link override Signal_Override/_ovrdval: Value=KOUTP_VMCSteerFaultRequest_enum_ovrdval
  VVMC_VehicleSpeed_kph_Inproc : FVT_lib/outp/OverrideAndLimit  SystemSampleTime=-1  VariantActivationTime=update diagram  Latency=0  AutoFrameSizeCalculation=off
      link override Signal_Limit/_maxval: Value=KOUTP_VehicleSpeed_kph_maxval
      link override Signal_Limit/_minval: Value=KOUTP_VehicleSpeed_kph_minval
      link override Signal_Override/_ovrdflg: Value=KOUTP_VehicleSpeed_kph_ovrdflg
      link override Signal_Override/_ovrdval: Value=KOUTP_VehicleSpeed_kph_ovrdval
  VVMC_VehicleSpeed_mph_Inproc : FVT_lib/outp/OverrideAndLimit  SystemSampleTime=-1  VariantActivationTime=update diagram  Latency=0  AutoFrameSizeCalculation=off
      link override Signal_Limit/_maxval: Value=KOUTP_VehicleSpeed_mph_maxval
      link override Signal_Limit/_minval: Value=KOUTP_VehicleSpeed_mph_minval
      link override Signal_Override/_ovrdflg: Value=KOUTP_VehicleSpeed_mph_ovrdflg
      link override Signal_Override/_ovrdval: Value=KOUTP_VehicleSpeed_mph_ovrdval
  VOUTP_HVTHCMSysAvail_enum : Outport
  VOUTP_LVBattVoltSta_enum : Outport  Port=2
  VOUTP_VehHVPwrAvail4THCM_W : Outport  Port=3
  VOUTP_VehSpeed_kph : Outport  Port=4
  VOUTP_VehSpeedTimeOut_flg : Outport  Port=5
  VOUTP_FSOffSw_enum : Outport  Port=6
  VOUTP_FSOffSwTimeOut_flg : Outport  Port=7
  VOUTP_ChrgPlugSta_enum : Outport  Port=8
  VOUTP_PASDRMR_cm : Outport  Port=9
  VOUTP_PASDRML_cm : Outport  Port=10
  VOUTP_PASDRCR_cm : Outport  Port=11
  VOUTP_PASDRCL_cm : Outport  Port=12
  VOUTP_PASDFMR_cm : Outport  Port=13
  VOUTP_PASDFML_cm : Outport  Port=14
  VOUTP_PASDFCR_cm : Outport  Port=15
  VOUTP_PASDFCL_cm : Outport  Port=16
  VOUTP_APSDRLR_cm : Outport  Port=17
  VOUTP_APSDRLL_cm : Outport  Port=18
  VOUTP_APSDFLR_cm : Outport  Port=19
  VOUTP_APSDFLL_cm : Outport  Port=20
  VOUTP_PASAFCL_enum : Outport  Port=21
  VOUTP_PASARMR_enum : Outport  Port=22
  VOUTP_PASARML_enum : Outport  Port=23
  VOUTP_PASARCR_enum : Outport  Port=24
  VOUTP_PASARCL_enum : Outport  Port=25
  VOUTP_PASAFMR_enum : Outport  Port=26
  VOUTP_PASAFML_enum : Outport  Port=27
  VOUTP_PASAFCR_enum : Outport  Port=28
  VOUTP_USSStaRMR_flg : Outport  Port=29
  VOUTP_USSStaRML_flg : Outport  Port=30
  VOUTP_USSStaRLR_flg : Outport  Port=31
  VOUTP_USSStaRLL_flg : Outport  Port=32
  VOUTP_USSStaRCR_flg : Outport  Port=33
  VOUTP_USSStaRCL_flg : Outport  Port=34
  VOUTP_USSStaFMR_flg : Outport  Port=35
  VOUTP_USSStaFML_flg : Outport  Port=36
  VOUTP_USSStaFLR_flg : Outport  Port=37
  VOUTP_USSStaFLL_flg : Outport  Port=38
  VOUTP_USSStaFCR_flg : Outport  Port=39
  VOUTP_USSStaFCL_flg : Outport  Port=40
  VOUTP_Chime_enum : Outport  Port=41
  VOUTP_SNSRLayout_enum : Outport  Port=42
  VOUTP_StaFSya_flg : Outport  Port=43
  VOUTP_ModOperation_enum : Outport  Port=44
  VOUTP_BrkPedalPos_pct : Outport  Port=45
  VOUTP_BrkPedalPosTimeOut_flg : Outport  Port=46
  VOUTP_LFRawWhlSpeed_kph : Outport  Port=47
  VOUTP_LFRawWhlSpeedTimeOut_flg : Outport  Port=48
  VOUTP_RFRawWhlSpeed_kph : Outport  Port=49
  VOUTP_RFRawWhlSpeedTimeOut_flg : Outport  Port=50
  VOUTP_LRRawWhlSpeed_kph : Outport  Port=51
  VOUTP_LRRawWhlSpeedTimeOut_flg : Outport  Port=52
  VOUTP_RRRawWhlSpeed_kph : Outport  Port=53
  VOUTP_RRRawWhlSpeedTimeOut_flg : Outport  Port=54
  VOUTP_LFRawWhlSpeedV_flg : Outport  Port=55
  VOUTP_LFRawWhlSpeedVTimeOut_flg : Outport  Port=56
  VOUTP_RFRawWhlSpeedV_flg : Outport  Port=57
  VOUTP_RFRawWhlSpeedVTimeOut_flg : Outport  Port=58
  VOUTP_LRRawWhlSpeedV_flg : Outport  Port=59
  VOUTP_LRRawWhlSpeedVTimeOut_flg : Outport  Port=60
  VOUTP_RRRawWhlSpeedV_flg : Outport  Port=61
  VOUTP_RRRawWhlSpeedVTimeOut_flg : Outport  Port=62
  VOUTP_LFWhlRotDir_enum : Outport  Port=63
  VOUTP_LFWhlRotDirTimeOut_flg : Outport  Port=64
  VOUTP_RFWhlRotDir_enum : Outport  Port=65
  VOUTP_RFWhlRotDirTimeOut_flg : Outport  Port=66
  VOUTP_LRWhlRotDir_enum : Outport  Port=67
  VOUTP_LRWhlRotDirTimeOut_flg : Outport  Port=68
  VOUTP_RRWhlRotDir_enum : Outport  Port=69
  VOUTP_RRWhlRotDirTimeOut_flg : Outport  Port=70
  VOUTP_LFPulseCountV_flg : Outport  Port=71
  VOUTP_LFPulseCountVTimeOut_flg : Outport  Port=72
  VOUTP_RFPulseCountV_flg : Outport  Port=73
  VOUTP_RFPulseCountVTimeOut_flg : Outport  Port=74
  VOUTP_LRPulseCountV_flg : Outport  Port=75
  VOUTP_LRPulseCountVTimeOut_flg : Outport  Port=76
  VOUTP_RRPulseCountV_flg : Outport  Port=77
  VOUTP_RRPulseCountVTimeOut_flg : Outport  Port=78
  VOUTP_LFPulseCount_enum : Outport  Port=79
  VOUTP_LFPulseCountTimeOut_flg : Outport  Port=80
  VOUTP_RFPulseCount_enum : Outport  Port=81
  VOUTP_RFPulseCountTimeOut_flg : Outport  Port=82
  VOUTP_LRPulseCount_enum : Outport  Port=83
  VOUTP_LRPulseCountTimeOut_flg : Outport  Port=84
  VOUTP_RRPulseCount_enum : Outport  Port=85
  VOUTP_RRPulseCountTimeOut_flg : Outport  Port=86
  VOUTP_ShifterHandleCmd_enum : Outport  Port=87
  VOUTP_ShifterHandleCmdTimeOut_flg : Outport  Port=88
  VOUTP_DriIntend_enum : Outport  Port=89
  VOUTP_DriIntendTimeOut_flg : Outport  Port=90
  VOUTP_EPSAOIControl_enum : Outport  Port=91
  VOUTP_EPSAOIControlTimeOut_flg : Outport  Port=92
  VOUTP_SASAngle_Deg : Outport  Port=93
  VOUTP_SASAngleTimeOut_flg : Outport  Port=94
  VOUTP_SASSpeed_degps : Outport  Port=95
  VOUTP_SASSpeedTimeOut_flg : Outport  Port=96
  VOUTP_SASSpeedValid_flg : Outport  Port=97
  VOUTP_SASSpeedValidTimeOut_flg : Outport  Port=98
  VOUTP_SASCAL_flg : Outport  Port=99
  VOUTP_SASCALTimeOut_flg : Outport  Port=100
  VOUTP_SASV_flg : Outport  Port=101
  VOUTP_SASVTimeOut_flg : Outport  Port=102
  VOUTP_GRADE_Deg : Outport  Port=103
  VOUTP_GRADETimeOut_flg : Outport  Port=104
  VOUTP_YawRate_degps : Outport  Port=105
  VOUTP_YawRateTimeOut_flg : Outport  Port=106
  VOUTP_LatAccel_Gps : Outport  Port=107
  VOUTP_LatAccelTimeOut_flg : Outport  Port=108
  VOUTP_LongAccel_Gps : Outport  Port=109
  VOUTP_LongAccelTimeOut_flg : Outport  Port=110
  VOUTP_MCPressure_bar : Outport  Port=111
  VOUTP_MCPressureTimeOut_flg : Outport  Port=112
  VOUTP_YawRateV_flg : Outport  Port=113
  VOUTP_YawRateVTimeOut_flg : Outport  Port=114
  VOUTP_LatAccelV_flg : Outport  Port=115
  VOUTP_LatAccelVTimeOut_flg : Outport  Port=116
  VOUTP_LongAccelV_flg : Outport  Port=117
  VOUTP_LongAccelVTimeOut_flg : Outport  Port=118
  VOUTP_MCPressureV_bar : Outport  Port=119
  VOUTP_MCPressureVTimeOut_flg : Outport  Port=120
  VOUTP_BrkSwSta_flg : Outport  Port=121
  VOUTP_BrkSwStaTimeOut_flg : Outport  Port=122
  VOUTP_BrkSwV_flg : Outport  Port=123
  VOUTP_BrkSwVTimeOut_flg : Outport  Port=124
  VOUTP_ESCStandstill_flg : Outport  Port=125
  VOUTP_ESCStandstillTimeOut_flg : Outport  Port=126
  VOUTP_ESCAPSSta_enum : Outport  Port=127
  VOUTP_ESCAPSStaTimeOut_flg : Outport  Port=128
  VOUTP_EPBExtReleaseAvail_flg : Outport  Port=129
  VOUTP_EPBExtReleaseAvailTimeOut_flg : Outport  Port=130
  VOUTP_EPBExtApplyAvail_flg : Outport  Port=131
  VOUTP_EPBExtApplyAvailTimeOut_flg : Outport  Port=132
  VOUTP_EPBErrSta_enum : Outport  Port=133
  VOUTP_EPBErrStaTimeOut_flg : Outport  Port=134
  VOUTP_EPBSta_enum : Outport  Port=135
  VOUTP_EPBStaTimeOut_flg : Outport  Port=136
  VOUTP_AVMparkingcancel_enum : Outport  Port=137
  VOUTP_AVMparkingcancelTimeOut_flg : Outport  Port=138
  VOUTP_AVMparkingexcute_enum : Outport  Port=139
  VOUTP_AVMparkingexcuteTimeOut_flg : Outport  Port=140
  VOUTP_AVMParkingmode_enum : Outport  Port=141
  VOUTP_AVMParkingmodeTimeOut_flg : Outport  Port=142
  VOUTP_AVMErrSTA_flg : Outport  Port=143
  VOUTP_AVMErrSTATimeOut_flg : Outport  Port=144
  VOUTP_IVIStatus_flg : Outport  Port=145
  VOUTP_IVIStatusTimeOut_flg : Outport  Port=146
  VOUTP_CAASSw_enum : Outport  Port=147
  VOUTP_CAASSwTimeOut_flg : Outport  Port=148
  VOUTP_IVIScreen_enum : Outport  Port=149
  VOUTP_IVIScreenTimeOut_flg : Outport  Port=150
  VOUTP_ABSActive_flg : Outport  Port=151
  VOUTP_ABSActiveTimeOut_flg : Outport  Port=152
  VOUTP_TCSActive_flg : Outport  Port=153
  VOUTP_TCSActiveTimeOut_flg : Outport  Port=154
  VOUTP_DriverSeatBeltCmd_flg : Outport  Port=155
  VOUTP_DriverSeatBeltCmdTimeOut_flg : Outport  Port=156
  VOUTP_APSProgressPCT_pct : Outport  Port=157
  VOUTP_APSRQDisplay_enum : Outport  Port=158
  VOUTP_APSSWVer_enum : Outport  Port=159
  VOUTP_APSHWVer_enum : Outport  Port=160
  VOUTP_APSExitCondition_enum : Outport  Port=161
  VOUTP_APSAngleTarget_Deg : Outport  Port=162
  VOUTP_APSVRqEPASCtrl_flg : Outport  Port=163
  VOUTP_APSRqEPASCtrl_flg : Outport  Port=164
  VOUTP_CAASSta_enum : Outport  Port=165
  VOUTP_AntitheftSta_enum : Outport  Port=166
  VOUTP_TailgateRemote_enum : Outport  Port=167
  VOUTP_HornCtrl_flg : Outport  Port=168
  VOUTP_AllDoorSW_flg : Outport  Port=169
  VOUTP_BCMDoorLockSta_flg : Outport  Port=170
  VOUTP_AntitheftSeatFlod_flg : Outport  Port=171
  VOUTP_HoodSW_flg : Outport  Port=172
  VOUTP_TailgateSW_flg : Outport  Port=173
  VOUTP_DrDoorSW_flg : Outport  Port=174
  VOUTP_PsDoorSW_flg : Outport  Port=175
  VOUTP_RLDoorSW_flg : Outport  Port=176
  VOUTP_RRDoorSW_flg : Outport  Port=177
  VOUTP_LockSetting_flg : Outport  Port=178
  VOUTP_FrChargingDoorCtrl_enum : Outport  Port=179
  VOUTP_RrChargingDoorCtrl_enum : Outport  Port=180
  VOUTP_CrashDetd_flg : Outport  Port=181
  VOUTP_CTDCtrl_enum : Outport  Port=182
  VOUTP_DoorLockIND_flg : Outport  Port=183
  VOUTP_CTDLockSW_flg : Outport  Port=184
  VOUTP_Dimmer_pct : Outport  Port=185
  VOUTP_DimmerEN_flg : Outport  Port=186
  VOUTP_PosLamp_flg : Outport  Port=187
  VOUTP_LBeam_flg : Outport  Port=188
  VOUTP_HBeam_flg : Outport  Port=189
  VOUTP_RrFogLamp_flg : Outport  Port=190
  VOUTP_BrakeLamp_flg : Outport  Port=191
  VOUTP_ReverseLamp_flg : Outport  Port=192
  VOUTP_LDRL_flg : Outport  Port=193
  VOUTP_RDRL_flg : Outport  Port=194
  VOUTP_LBSD_flg : Outport  Port=195
  VOUTP_RBSD_flg : Outport  Port=196
  VOUTP_HazardSW_flg : Outport  Port=197
  VOUTP_LTurnLP_flg : Outport  Port=198
  VOUTP_RTurnLP_flg : Outport  Port=199
  VOUTP_BCMBuzzerReq_flg : Outport  Port=200
  VOUTP_MirrorCtrl_enum : Outport  Port=201
  VOUTP_MirrorDefog_flg : Outport  Port=202
  VOUTP_RrDefog_flg : Outport  Port=203
  VOUTP_RoomLampH_flg : Outport  Port=204
  VOUTP_RoomLampL_flg : Outport  Port=205
  VOUTP_TrunkRel_flg : Outport  Port=206
  VOUTP_TailgateHDSW_flg : Outport  Port=207
  VOUTP_FrWiperL_flg : Outport  Port=208
  VOUTP_FrWiperH_flg : Outport  Port=209
  VOUTP_RrWiper_flg : Outport  Port=210
  VOUTP_WasherCtrl_enum : Outport  Port=211
  VOUTP_WiperFixMode_flg : Outport  Port=212
  VOUTP_AmbLightBreath1_enum : Outport  Port=213
  VOUTP_AmbLightBreath2_enum : Outport  Port=214
  VOUTP_AmbLightBreath3_enum : Outport  Port=215
  VOUTP_AmbLightBreath4_enum : Outport  Port=216
  VOUTP_AmbLightBreath5_enum : Outport  Port=217
  VOUTP_AmbLightBreath6_enum : Outport  Port=218
  VOUTP_AmbLightBrightness1_enum : Outport  Port=219
  VOUTP_AmbLightBrightness2_enum : Outport  Port=220
  VOUTP_AmbLightBrightness3_enum : Outport  Port=221
  VOUTP_AmbLightBrightness4_enum : Outport  Port=222
  VOUTP_AmbLightBrightness5_enum : Outport  Port=223
  VOUTP_AmbLightBrightness6_enum : Outport  Port=224
  VOUTP_AmbLightColor1_enum : Outport  Port=225
  VOUTP_AmbLightColor2_enum : Outport  Port=226
  VOUTP_AmbLightColor3_enum : Outport  Port=227
  VOUTP_AmbLightColor4_enum : Outport  Port=228
  VOUTP_AmbLightColor5_enum : Outport  Port=229
  VOUTP_AmbLightColor6_enum : Outport  Port=230
  VOUTP_LampPwr_flg : Outport  Port=231
  VOUTP_SPTGDet_flg : Outport  Port=232
  VOUTP_APSOpenPTG_flg : Outport  Port=233
  VOUTP_FollowMe_flg : Outport  Port=234
  VOUTP_IVIRST_flg : Outport  Port=235
  VOUTP_CountAlarm_enum : Outport  Port=236
  VOUTP_MFSWTri_flg : Outport  Port=237
  VOUTP_MirrorFlodPos_flg : Outport  Port=238
  VOUTP_FuelDoorPos_flg : Outport  Port=239
  VOUTP_MFRDNBrightReq_pct : Outport  Port=240
  VOUTP_RoomLampMode_flg : Outport  Port=241
  VOUTP_IVIPTGUSStaSW_flg : Outport  Port=242
  VOUTP_PTGInnerSW2_enum : Outport  Port=243
  VOUTP_LDrvCtrlCmd_pct : Outport  Port=244
  VOUTP_LPasCtrlCmd_pct : Outport  Port=245
  VOUTP_LRLDCtrlCmd_pct : Outport  Port=246
  VOUTP_LRRDCtrlCmd_pct : Outport  Port=247
  VOUTP_APMDoorControlSta_flg : Outport  Port=248
  VOUTP_AmbFunEN_flg : Outport  Port=249
  VOUTP_AmbWelEN_flg : Outport  Port=250
  VOUTP_AmbDimEN_flg : Outport  Port=251
  VOUTP_AmbLinkDriSta_flg : Outport  Port=252
  VOUTP_AmbPwrWarnEN_flg : Outport  Port=253
  VOUTP_AmbODAEN_flg : Outport  Port=254
  VOUTP_AmbColorSta_enum : Outport  Port=255
  VOUTP_AmbBrightSta_enum : Outport  Port=256
  VOUTP_LockAlarm_enum : Outport  Port=257
  VOUTP_ATCtrl_enum : Outport  Port=258
  VOUTP_fUnlockSingle_flg : Outport  Port=259
  VOUTP_UserNow_enum : Outport  Port=260
  VOUTP_AmbFunENFlash_enum : Outport  Port=261
  VOUTP_AmbWelENFlash_enum : Outport  Port=262
  VOUTP_AmbDimENFlash_enum : Outport  Port=263
  VOUTP_AmbLinkDriStaFlash_enum : Outport  Port=264
  VOUTP_AmbPwrWarnENFlash_enum : Outport  Port=265
  VOUTP_AmbODAENFlash_enum : Outport  Port=266
  VOUTP_AmbColorSta1_enum : Outport  Port=267
  VOUTP_AmbColorSta2_enum : Outport  Port=268
  VOUTP_AmbColorSta3_enum : Outport  Port=269
  VOUTP_AmbColorSta4_enum : Outport  Port=270
  VOUTP_AmbColorSta5_enum : Outport  Port=271
  VOUTP_AmbColorSta7_enum : Outport  Port=272
  VOUTP_AmbBrightnessSta1_enum : Outport  Port=273
  VOUTP_AmbBrightnessSta2_enum : Outport  Port=274
  VOUTP_AmbBrightnessSta3_enum : Outport  Port=275
  VOUTP_AmbBrightnessSta4_enum : Outport  Port=276
  VOUTP_AmbBrightnessSta5_enum : Outport  Port=277
  VOUTP_AmbBrightnessSta7_enum : Outport  Port=278
  VOUTP_HazardIND_flg : Outport  Port=279
  VOUTP_DimSwSta_flg : Outport  Port=280
  VOUTP_PassSWSta_flg : Outport  Port=281
  VOUTP_FWipSwSta_enum : Outport  Port=282
  VOUTP_FWasSwSta_enum : Outport  Port=283
  VOUTP_TurnSwSta_enum : Outport  Port=284
  VOUTP_ActAPSPosn_pct : Outport  Port=285
  VOUTP_EAPS1MIN_pct : Outport  Port=286
  VOUTP_EAPS2MIN_pct : Outport  Port=287
  VOUTP_DKCTimeSN_cnt : Outport  Port=288
  VOUTP_DKCAuthSta_enum : Outport  Port=289
  VOUTP_DISCTurn_flg : Outport  Port=290
  VOUTP_DISCTargetSpd_kph : Outport  Port=291
  VOUTP_DISCSta_enum : Outport  Port=292
  VOUTP_DISCButtSta_flg : Outport  Port=293
  VOUTP_AllCANTxReq_flg : Outport  Port=294
  VOUTP_NMmTxReq_flg : Outport  Port=295
  VOUTP_Awake_enum : Outport  Port=296
  VOUTP_CSB_flg : Outport  Port=297
  VOUTP_ErrorState_enum : Outport  Port=298
  VOUTP_NodeID_enum : Outport  Port=299
  VOUTP_PNI_flg : Outport  Port=300
  VOUTP_RptMsgReq_flg : Outport  Port=301
  VOUTP_WakeUp_enum : Outport  Port=302
  VOUTP_ActiveWU_flg : Outport  Port=303
  VOUTP_SysNMmSta_enum : Outport  Port=304
  VOUTP_NetworkReq_flg : Outport  Port=305
  VOUTP_PowerUpState_enum : Outport  Port=306
  VOUTP_PowerDownState_enum : Outport  Port=307
  VOUTP_PowerUpFault_enum : Outport  Port=308
  VOUTP_PowerDownFault_enum : Outport  Port=309
  VOUTP_ActiveDischargeReq_flg : Outport  Port=310
  VOUTP_DCDCEnaReq_flg : Outport  Port=311
  VOUTP_DCDCVoltSetpoint_V : Outport  Port=312
  VOUTP_HVBatCnctReq_flg : Outport  Port=313
  VOUTP_HVSysReadyToCharge_enum : Outport  Port=314
  VOUTP_PowerSta_enum : Outport  Port=315
  VOUTP_LVPwrSta_flg : Outport  Port=316
  VOUTP_HVPwrSta_flg : Outport  Port=317
  VOUTP_SysPowerMode_enum : Outport  Port=318
  VOUTP_FrMCUEnaReq_flg : Outport  Port=319
  VOUTP_RrMCUEnaReq_flg : Outport  Port=320
  VOUTP_DrivetrainSelect_enum : Outport  Port=321
  VOUTP_DrSeatSta_enum : Outport  Port=322
  VOUTP_PwrStaSelect_enum : Outport  Port=323
  VOUTP_PwrStaConstraint_enum : Outport  Port=324
  VOUTP_TCountSta_enum : Outport  Port=325
  VOUTP_PwrUpReq_enum : Outport  Port=326
  VOUTP_PwrDownReq_enum : Outport  Port=327
  VOUTP_LowSOCWarn_enum : Outport  Port=328
  VOUTP_ReVehThdChkSta_enum : Outport  Port=329
  VOUTP_LVSysErrPwrOutErr_flg : Outport  Port=330
  VOUTP_EvccAplusPwrUpReq_flg : Outport  Port=331
  VOUTP_PwrStaONTOPopReq_flg : Outport  Port=332
  VOUTP_IVIPwrStaONTOPopT_s : Outport  Port=333
  VOUTP_LVChrgHoldTtimer_s : Outport  Port=334
  VOUTP_LVBattChrgTimeCnt_s : Outport  Port=335
  VOUTP_SilentChkAllowSleep_flg : Outport  Port=336
  VOUTP_TimerAllowSleep_flg : Outport  Port=337
  VOUTP_FDADC12VDetAvg_mV : Outport  Port=338
  VOUTP_PMMAllowECUSleep_flg : Outport  Port=339
  VOUTP_LVSilentChrgSta_enum : Outport  Port=340
  VOUTP_LVSilentChrgReq_flg : Outport  Port=341
  VOUTP_LVSilentChrgLv_enum : Outport  Port=342
  VOUTP_CtrlFrPwrStbA1P_flg : Outport  Port=343
  VOUTP_CtrlFrRC1_flg : Outport  Port=344
  VOUTP_CtrlFrBMSCCUCIR_flg : Outport  Port=345
  VOUTP_CtrlFrEDUINVERTER_flg : Outport  Port=346
  VOUTP_HWResetSta_enum : Outport  Port=347
  VOUTP_CtrlDrPwrStbA2_flg : Outport  Port=348
  VOUTP_PwrStaTOSta_enum : Outport  Port=349
  VOUTP_Sched_ChgTOSta_enum : Outport  Port=350
  VOUTP_PwrReq_OTA_enum : Outport  Port=351
  VOUTP_OTAPwrReqOFFChkSta_enum : Outport  Port=352
  VOUTP_OTAPwrReqStdChkSta_enum : Outport  Port=353
  VOUTP_HWVer1_cnt : Outport  Port=354
  VOUTP_HWVer2_cnt : Outport  Port=355
  VOUTP_HWVer3_cnt : Outport  Port=356
  VOUTP_CarModel1_cnt : Outport  Port=357
  VOUTP_CarModel2_cnt : Outport  Port=358
  VOUTP_CarModel3_cnt : Outport  Port=359
  VOUTP_ECU1_cnt : Outport  Port=360
  VOUTP_ECU2_cnt : Outport  Port=361
  VOUTP_Major1_cnt : Outport  Port=362
  VOUTP_Major2_cnt : Outport  Port=363
  VOUTP_Minor1_cnt : Outport  Port=364
  VOUTP_Minor2_cnt : Outport  Port=365
  VOUTP_Patch1_cnt : Outport  Port=366
  VOUTP_Patch2_cnt : Outport  Port=367
  VOUTP_Country1_cnt : Outport  Port=368
  VOUTP_Country2_cnt : Outport  Port=369
  VOUTP_Variation_cnt : Outport  Port=370
  VOUTP_Dash1_cnt : Outport  Port=371
  VOUTP_Change1_cnt : Outport  Port=372
  VOUTP_Change2_cnt : Outport  Port=373
  VOUTP_Dash2_cnt : Outport  Port=374
  VOUTP_SHA1_cnt : Outport  Port=375
  VOUTP_SHA2_cnt : Outport  Port=376
  VOUTP_SHA3_cnt : Outport  Port=377
  VOUTP_SHA4_cnt : Outport  Port=378
  VOUTP_SHA5_cnt : Outport  Port=379
  VOUTP_SHA6_cnt : Outport  Port=380
  VOUTP_SHA7_cnt : Outport  Port=381
  VOUTP_SHA8_cnt : Outport  Port=382
  VOUTP_NvWriteReqRisingEdge_flg : Outport  Port=383
  VOUTP_FdcSlpReqRisingEdge_flg : Outport  Port=384
  VOUTP_FdcSlpTime_sec : Outport  Port=385
  VOUTP_PmicBootReason_enum : Outport  Port=386
  VOUTP_WisrBootReason_raw32 : Outport  Port=387
  VOUTP_AcoreRebootCmdACK_flg : Outport  Port=388
  VOUTP_CurrentNmState_enum : Outport  Port=389
  VOUTP_FDCompCmd_rpm : Outport  Port=390
  VOUTP_FDSOV1Cmd_flg : Outport  Port=391
  VOUTP_FDSOV2Cmd_flg : Outport  Port=392
  VOUTP_FDSOV3Cmd_flg : Outport  Port=393
  VOUTP_FDEXV1Cmd_step : Outport  Port=394
  VOUTP_FDEXV2Cmd_step : Outport  Port=395
  VOUTP_FDSOTXVCmd_flg : Outport  Port=396
  VOUTP_FDFWVCmd_flg : Outport  Port=397
  VOUTP_FDTWVCmd_pct : Outport  Port=398
  VOUTP_FDFrWPTCHeatPwrCmd_W : Outport  Port=399
  VOUTP_CoolgFanActDuty_pct : Outport  Port=400
  VOUTP_FDAGSCmd_enum : Outport  Port=401
  VOUTP_FDEWP1Cmd_enum : Outport  Port=402
  VOUTP_FDEWP2Cmd_enum : Outport  Port=403
  VOUTP_FDEWP3Cmd_enum : Outport  Port=404
  VOUTP_FDFrLeAPTCHeatPwrCmd_W : Outport  Port=405
  VOUTP_FDFrRiAPTCHeatPwrCmd_W : Outport  Port=406
  VOUTP_FDRrAPTCHeatPwrCmd_W : Outport  Port=407
  VOUTP_FDBlowerCmd_pct : Outport  Port=408
  VOUTP_BatteryMode_enum : Outport  Port=409
  VOUTP_EDriveMode_enum : Outport  Port=410
  VOUTP_CabinMode_enum : Outport  Port=411
  VOUTP_CCUACLampSts_flg : Outport  Port=412
  VOUTP_CCUAutoLampSts_flg : Outport  Port=413
  VOUTP_CCUACMaxLampSts_flg : Outport  Port=414
  VOUTP_CCUSyncLampSts_flg : Outport  Port=415
  VOUTP_sigAirIntenZon1St_enum : Outport  Port=416
  VOUTP_sigWindDirZon1St_enum : Outport  Port=417
  VOUTP_sigRecircSt_flg : Outport  Port=418
  VOUTP_sigSetTempZon1St_C : Outport  Port=419
  VOUTP_sigSetTempZon2St_C : Outport  Port=420
  VOUTP_sigClntTHvBattOut_C : Outport  Port=421
  VOUTP_sigCbnSolarLeft_W : Outport  Port=422
  VOUTP_sigClntTHvBattIn_C : Outport  Port=423
  VOUTP_sigCbnSolarRight_W : Outport  Port=424
  VOUTP_sigAmbAirT_C : Outport  Port=425
  VOUTP_sigCbnAirT_C : Outport  Port=426
  VOUTP_ACSubMode_enum : Outport  Port=427
  VOUTP_FDRecyAutoCmd_enum : Outport  Port=428
  VOUTP_ACModeMem_enum : Outport  Port=429
  VOUTP_Face_flg : Outport  Port=430
  VOUTP_Foot_flg : Outport  Port=431
  VOUTP_Frost_flg : Outport  Port=432
  VOUTP_FaceM_flg : Outport  Port=433
  VOUTP_FootM_flg : Outport  Port=434
  VOUTP_CCUSyncSts_flg : Outport  Port=435
  VOUTP_ACForceOFF_flg : Outport  Port=436
  VOUTP_RecAutoFlg_flg : Outport  Port=437
  VOUTP_AirIntenZone1M_enum : Outport  Port=438
  VOUTP_fdefog_flg : Outport  Port=439
  VOUTP_sigSetTempZon2StM_C : Outport  Port=440
  VOUTP_FDCTHCMAPTCWarningSta_flg : Outport  Port=441
  VOUTP_LFBatWarn_flg : Outport  Port=442
  VOUTP_RFBatWarn_flg : Outport  Port=443
  VOUTP_LRBatWarn_flg : Outport  Port=444
  VOUTP_RRBatWarn_flg : Outport  Port=445
  VOUTP_LFWheelPress_raw8 : Outport  Port=446
  VOUTP_RFWheelPress_raw8 : Outport  Port=447
  VOUTP_LRWheelPress_raw8 : Outport  Port=448
  VOUTP_RRWheelPress_raw8 : Outport  Port=449
  VOUTP_LFWheelTemp_C : Outport  Port=450
  VOUTP_RFWheelTemp_C : Outport  Port=451
  VOUTP_LRWheelTemp_C : Outport  Port=452
  VOUTP_RRWheelTemp_C : Outport  Port=453
  VOUTP_LFSensorFail_flg : Outport  Port=454
  VOUTP_RFSensorFail_flg : Outport  Port=455
  VOUTP_LRSensorFail_flg : Outport  Port=456
  VOUTP_RRSensorFail_flg : Outport  Port=457
  VOUTP_LFWheelDebug_flg : Outport  Port=458
  VOUTP_LRWheelDebug_flg : Outport  Port=459
  VOUTP_RFWheelDebug_flg : Outport  Port=460
  VOUTP_RRWheelDebug_flg : Outport  Port=461
  VOUTP_TPMSResButtAllow_flg : Outport  Port=462
  VOUTP_TPMSCaliButtAllow_flg : Outport  Port=463
  VOUTP_LFPressIndi_enum : Outport  Port=464
  VOUTP_RFPressIndi_enum : Outport  Port=465
  VOUTP_LRPressIndi_enum : Outport  Port=466
  VOUTP_RRPressIndi_enum : Outport  Port=467
  VOUTP_TPMSWarnIndi_enum : Outport  Port=468
  VOUTP_LFWheelTmpIndi_flg : Outport  Port=469
  VOUTP_RFWheelTmpIndi_flg : Outport  Port=470
  VOUTP_LRWheelTmpIndi_flg : Outport  Port=471
  VOUTP_RRWheelTmpIndi_flg : Outport  Port=472
  VOUTP_LFWheelPSW_raw8 : Outport  Port=473
  VOUTP_LRWheelPSW_raw8 : Outport  Port=474
  VOUTP_RFWheelPSW_raw8 : Outport  Port=475
  VOUTP_RRWheelPSW_raw8 : Outport  Port=476
  VOUTP_CWheelTips_enum : Outport  Port=477
  VOUTP_AutoLTips_enum : Outport  Port=478
  VOUTP_LFSensorMode_flg : Outport  Port=479
  VOUTP_RFSensorMode_flg : Outport  Port=480
  VOUTP_LRSensorMode_flg : Outport  Port=481
  VOUTP_RRSensorMode_flg : Outport  Port=482
  VOUTP_S1ID_raw32 : Outport  Port=483
  VOUTP_S2ID_raw32 : Outport  Port=484
  VOUTP_S3ID_raw32 : Outport  Port=485
  VOUTP_S4ID_raw32 : Outport  Port=486
  VOUTP_S1L_enum : Outport  Port=487
  VOUTP_S2L_enum : Outport  Port=488
  VOUTP_S3L_enum : Outport  Port=489
  VOUTP_S4L_enum : Outport  Port=490
  VOUTP_ALFin_flg : Outport  Port=491
  VOUTP_LFP20_raw8 : Outport  Port=492
  VOUTP_RFP20_raw8 : Outport  Port=493
  VOUTP_LRP20_raw8 : Outport  Port=494
  VOUTP_RRP20_raw8 : Outport  Port=495
  VOUTP_FAT_flg : Outport  Port=496
  VOUTP_IDin_raw32 : Outport  Port=497
  VOUTP_S1WheelDebugALTU_pct : Outport  Port=498
  VOUTP_S2WheelDebugALTU_pct : Outport  Port=499
  VOUTP_S3WheelDebugALTU_pct : Outport  Port=500
  VOUTP_S4WheelDebugALTU_pct : Outport  Port=501
  VOUTP_ID1messageALTU_raw8 : Outport  Port=502
  VOUTP_ID2messageALTU_raw8 : Outport  Port=503
  VOUTP_ID3messageALTU_raw8 : Outport  Port=504
  VOUTP_ID4messageALTU_raw8 : Outport  Port=505
  VOUTP_Chkfin_flg : Outport  Port=506
  VOUTP_SetIDLoc_flg : Outport  Port=507
  VOUTP_TPMSStorge_flg : Outport  Port=508
  VOUTP_ChkStorge_flg : Outport  Port=509
  VOUTP_TPMSResButt_flg : Outport  Port=510
  VOUTP_LFPindi_enum : Outport  Port=511
  VOUTP_RFPind_enum : Outport  Port=512
  VOUTP_LRPindi_enum : Outport  Port=513
  VOUTP_RRPindi_enum : Outport  Port=514
  VOUTP_WriteChkLFID_raw : Outport  Port=515
  VOUTP_WriteChkRFID_raw : Outport  Port=516
  VOUTP_WriteChkLRID_raw : Outport  Port=517
  VOUTP_WriteChkRRID_raw : Outport  Port=518
  VOUTP_WriteChkfinLFID_raw : Outport  Port=519
  VOUTP_WriteChkfinRFID_raw : Outport  Port=520
  VOUTP_WriteChkfinLRID_raw : Outport  Port=521
  VOUTP_WriteChkfinRRID_raw : Outport  Port=522
  VOUTP_Flashchkdatavalid_enum : Outport  Port=523
  VOUTP_Flashdatavalid_enum : Outport  Port=524
  VOUTP_unlearnSfali_flg : Outport  Port=525
  VOUTP_unlearnSfailvalid_enum : Outport  Port=526
  VOUTP_Prepresstempvalid_enum : Outport  Port=527
  VOUTP_FlashS1ID_raw : Outport  Port=528
  VOUTP_FlashS2ID_raw : Outport  Port=529
  VOUTP_FlashS3ID_raw : Outport  Port=530
  VOUTP_FlashS4ID_raw : Outport  Port=531
  VOUTP_FlashIDvalid_enum : Outport  Port=532
  VOUTP_ParkRequest_flg : Outport  Port=533
  VOUTP_TqSourceFr_enum : Outport  Port=534
  VOUTP_TqSourceRr_enum : Outport  Port=535
  VOUTP_FrEDUAvailBrkRgnTq_Nm : Outport  Port=536
  VOUTP_RrEDUAvailBrkRgnTq_Nm : Outport  Port=537
  VOUTP_EVDriveMode_enum : Outport  Port=538
  VOUTP_ShiftGearPosn_enum : Outport  Port=539
  VOUTP_PButtonSta_enum : Outport  Port=540
  VOUTP_FrActvDmpDisabReq_flg : Outport  Port=541
  VOUTP_RrActvDmpDisabReq_flg : Outport  Port=542
  VOUTP_FrRgnDecrSta_flg : Outport  Port=543
  VOUTP_RrRgnDecrSta_flg : Outport  Port=544
  VOUTP_DriverWhlTqDemFr_Nm : Outport  Port=545
  VOUTP_DriverWhlTqDemRr_Nm : Outport  Port=546
  VOUTP_FrEDUActTq_Nm : Outport  Port=547
  VOUTP_RrEDUActTq_Nm : Outport  Port=548
  VOUTP_FrEDURolRgnTq_Nm : Outport  Port=549
  VOUTP_RrEDURolRgnTq_Nm : Outport  Port=550
  VOUTP_FrEDUSpd_rpm : Outport  Port=551
  VOUTP_RrEDUSpd_rpm : Outport  Port=552
  VOUTP_FrEDUSpdValid_flg : Outport  Port=553
  VOUTP_FrEDUAvailBrkRgnTqV_flg : Outport  Port=554
  VOUTP_RrEDUSpdValid_flg : Outport  Port=555
  VOUTP_RrEDUAvailBrkRgnTqV_flg : Outport  Port=556
  VOUTP_RgnAbnorSta_flg : Outport  Port=557
  VOUTP_PTCSPermSta_flg : Outport  Port=558
  VOUTP_FrRgnPermSta_flg : Outport  Port=559
  VOUTP_RrRgnPermSta_flg : Outport  Port=560
  VOUTP_FrIdcMin_A : Outport  Port=561
  VOUTP_FrIdcMax_A : Outport  Port=562
  VOUTP_FrUdcMin_V : Outport  Port=563
  VOUTP_FrUdcMax_V : Outport  Port=564
  VOUTP_RrIdcMin_A : Outport  Port=565
  VOUTP_RrIdcMax_A : Outport  Port=566
  VOUTP_RrUdcMin_V : Outport  Port=567
  VOUTP_RrUdcMax_V : Outport  Port=568
  VOUTP_ReBrakeLPReq_flg : Outport  Port=569
  VOUTP_CreepON_flg : Outport  Port=570
  VOUTP_EquivAccPedalSWSta_flg : Outport  Port=571
  VOUTP_DriveProtEn_flg : Outport  Port=572
  VOUTP_ActParkRequest_flg : Outport  Port=573
  VOUTP_IVIPwrLockSta_enum : Outport  Port=574
  VOUTP_OPDHoldLamp_flg : Outport  Port=575
  VOUTP_SaveRegenMode_enum : Outport  Port=576
  VOUTP_FDCVCURegenMode_enum : Outport  Port=577
  VOUTP_SpdCtrlMode_enum : Outport  Port=578
  VOUTP_SpdCtrlSta_flg : Outport  Port=579
  VOUTP_SetSpd_kph : Outport  Port=580
  VOUTP_FrTMTqReq_Nm : Outport  Port=581
  VOUTP_RrTMTqReq_Nm : Outport  Port=582
  VOUTP_ReqOBCV2LEna_enum : Outport  Port=583
  VOUTP_ReqV2LIVIPopup_enum : Outport  Port=584
  VOUTP_FeatSetSpdFinal_raw32 : Outport  Port=585
  VOUTP_VehicleSpeed_mph : Outport  Port=586
  VOUTP_VehicleSpeed_kph : Outport  Port=587
  VOUTP_MeterIndSpeed_raw32 : Outport  Port=588
  VOUTP_VMCAEBCtrlAvail_flg : Outport  Port=589
  VOUTP_VMCACCCtrlAvail_flg : Outport  Port=590
  VOUTP_VMCCCCtrlAvail_flg : Outport  Port=591
  VOUTP_VMCMSACtrlAvail_flg : Outport  Port=592
  VOUTP_FeatArbitrSta_enum : Outport  Port=593
  VOUTP_FeatReqSpd_kph : Outport  Port=594
  VOUTP_JerkPCT_pct : Outport  Port=595
  VOUTP_LimitPCT_pct : Outport  Port=596
  VOUTP_FrontRearSlipRatioCtrl_flg : Outport  Port=597
  VOUTP_RearWhlSlipRatioCtrl_flg : Outport  Port=598
  VOUTP_SingleWhlSlipRatioCtrl_flg : Outport  Port=599
  VOUTP_LatAccCtrl_flg : Outport  Port=600
  VOUTP_SafetyCtrl_flg : Outport  Port=601
  VOUTP_SPD2ACCAct_flg : Outport  Port=602
  VOUTP_AccCalcuPID_mps2 : Outport  Port=603
  VOUTP_ISOAccLimit_mps2 : Outport  Port=604
  VOUTP_ISODecLimit_mps2 : Outport  Port=605
  VOUTP_ISOJerkLimit_mps3 : Outport  Port=606
  VOUTP_ACCRequiredAccel_mps2 : Outport  Port=607
  VOUTP_DISCReqAcc_mps2 : Outport  Port=608
  VOUTP_FeatArbitrFinal_enum : Outport  Port=609
  VOUTP_LateralCtrl_flg : Outport  Port=610
  VOUTP_ADASLKASta_enum : Outport  Port=611
  VOUTP_LKAStrToqReq_Nm : Outport  Port=612
  VOUTP_LKATOIFault_flg : Outport  Port=613
  VOUTP_LKATOIAct_enum : Outport  Port=614
  VOUTP_ADASAEBReq_enum : Outport  Port=615
  VOUTP_ADASFaultSta_flg : Outport  Port=616
  VOUTP_AEBVehHoldReq_flg : Outport  Port=617
  VOUTP_ACCVehHoldReq_flg : Outport  Port=618
  VOUTP_ADASDBSReq_enum : Outport  Port=619
  VOUTP_ADASACCSta_enum : Outport  Port=620
  VOUTP_ACCObjDist_m : Outport  Port=621
  VOUTP_ACCObjRelSpd_mps : Outport  Port=622
  VOUTP_TimeGapLevel_enum : Outport  Port=623
  VOUTP_ACCJerkUpperLimit_mps3 : Outport  Port=624
  VOUTP_ACCComfortBandUpper_mps2 : Outport  Port=625
  VOUTP_ACCJerkLowerLimit_mps3 : Outport  Port=626
  VOUTP_ACCComfortBandLower_mps2 : Outport  Port=627
  VOUTP_ADASVehSpdLim_raw32 : Outport  Port=628
  VOUTP_ADASShftPosnReqA_flg : Outport  Port=629
  VOUTP_ADASShftPosnReq_enum : Outport  Port=630
  VOUTP_ADASForceIdle_flg : Outport  Port=631
  VOUTP_HazardWarningReq_flg : Outport  Port=632
  VOUTP_RightTurnLightReq_flg : Outport  Port=633
  VOUTP_LeftTurnLightReq_flg : Outport  Port=634
  VOUTP_ADASFCWSta_enum : Outport  Port=635
  VOUTP_ADASLDWSta_enum : Outport  Port=636
  VOUTP_ADASFltWrnReq_flg : Outport  Port=637
  VOUTP_ACCObjDstLvl_enum : Outport  Port=638
  VOUTP_ForceLowBeam_enum : Outport  Port=639
  VOUTP_ACCTakeoverReq_flg : Outport  Port=640
  VOUTP_ADASWarningMsg_enum : Outport  Port=641
  VOUTP_ADASCAMSpdLim_enum : Outport  Port=642
  VOUTP_TargetType_enum : Outport  Port=643
  VOUTP_ADASSLIFSpdLim_enum : Outport  Port=644
  VOUTP_LKAHODDisplayWarning_flg : Outport  Port=645
  VOUTP_LKAHODSoundWarning_flg : Outport  Port=646
  VOUTP_ADASLFCSta_enum : Outport  Port=647
  VOUTP_ADASLaneModeL_enum : Outport  Port=648
  VOUTP_ADASLaneModeR_enum : Outport  Port=649
  VOUTP_ADASSLIFSta_enum : Outport  Port=650
  VOUTP_ADASISASta_enum : Outport  Port=651
  VOUTP_ADASLDWMute_flg : Outport  Port=652
  VOUTP_ADASFCWMute_flg : Outport  Port=653
  VOUTP_ADASLFCHandsOffWarning_enum : Outport  Port=654
  VOUTP_LVDADisabled_flg : Outport  Port=655
  VOUTP_LVDAMuteSta_enum : Outport  Port=656
  VOUTP_LVDAFailinfo_flg : Outport  Port=657
  VOUTP_LVDAWarning_flg : Outport  Port=658
  VOUTP_LVDAACCStatusInformation_flg : Outport  Port=659
  VOUTP_ADASLFCWarnSound_enum : Outport  Port=660
  VOUTP_FCMACCmode_enum : Outport  Port=661
  VOUTP_ADASLanetypeR_enum : Outport  Port=662
  VOUTP_ADASLanetypeL_enum : Outport  Port=663
  VOUTP_ADASLanecurveL_raw32 : Outport  Port=664
  VOUTP_ADASLanecurveR_raw32 : Outport  Port=665
  VOUTP_ADASAEBSta_enum : Outport  Port=666
  VOUTP_FCMLDWRequest_enum : Outport  Port=667
  VOUTP_FCMLDWFault_flg : Outport  Port=668
  VOUTP_ACCCtrlAvail_flg : Outport  Port=669
  VOUTP_ACCPedalOvrd_flg : Outport  Port=670
  VOUTP_TimeGapCalcu_s : Outport  Port=671
  VOUTP_CCCtrlSta_enum : Outport  Port=672
  VOUTP_MSACtrlSta_enum : Outport  Port=673
  VOUTP_APSCtrlAvail_flg : Outport  Port=674
  VOUTP_APSStaSys_enum : Outport  Port=675
  VOUTP_APSDecReqA_flg : Outport  Port=676
  VOUTP_APSDecReq_mps2 : Outport  Port=677
  VOUTP_APSReq_enum : Outport  Port=678
  VOUTP_CCMSASpdWar_flg : Outport  Port=679
  VOUTP_IMUEnaCmd_flg : Outport  Port=680
  VOUTP_CAASCtrlAvail_flg : Outport  Port=681
  VOUTP_CAASActive_flg : Outport  Port=682
  VOUTP_VMCRWSActvSta_enum : Outport  Port=683
  VOUTP_VMCRWSDfctvSta_enum : Outport  Port=684
  VOUTP_VMCRWSPositionReq_mm : Outport  Port=685
  VOUTP_VMCSteerFaultRequest_enum : Outport  Port=686
  wires:
  VACC_HVTHCMSysAvail_enum/1 -> VACC_HVTHCMSysAvail_enum_Inproc/1  "VACC_HVTHCMSysAvail_enum"
  VACC_HVTHCMSysAvail_enum_Inproc/1 -> UnitConverter1/1
  UnitConverter1/1 -> VOUTP_HVTHCMSysAvail_enum/1  "VOUTP_HVTHCMSysAvail_enum"
  VACC_LVBattVoltSta_enum/1 -> VACC_LVBattVoltSta_enum_Inproc/1  "VACC_LVBattVoltSta_enum"
  VACC_LVBattVoltSta_enum_Inproc/1 -> UnitConverter2/1
  UnitConverter2/1 -> VOUTP_LVBattVoltSta_enum/1  "VOUTP_LVBattVoltSta_enum"
  VACC_VehHVPwrAvail4THCM_W/1 -> VACC_VehHVPwrAvail4THCM_W_Inproc/1  "VACC_VehHVPwrAvail4THCM_W"
  VACC_VehHVPwrAvail4THCM_W_Inproc/1 -> UnitConverter3/1
  UnitConverter3/1 -> VOUTP_VehHVPwrAvail4THCM_W/1  "VOUTP_VehHVPwrAvail4THCM_W"
  VAPM_VehSpeed_kph/1 -> VAPM_VehSpeed_kph_Inproc/1  "VAPM_VehSpeed_kph"
  VAPM_VehSpeed_kph_Inproc/1 -> UnitConverter4/1
  UnitConverter4/1 -> VOUTP_VehSpeed_kph/1  "VOUTP_VehSpeed_kph"
  VAPM_VehSpeedTimeOut_flg/1 -> VAPM_VehSpeedTimeOut_flg_Inproc/1  "VAPM_VehSpeedTimeOut_flg"
  VAPM_VehSpeedTimeOut_flg_Inproc/1 -> UnitConverter5/1
  UnitConverter5/1 -> VOUTP_VehSpeedTimeOut_flg/1  "VOUTP_VehSpeedTimeOut_flg"
  VAPM_FSOffSw_enum/1 -> VAPM_FSOffSw_enum_Inproc/1  "VAPM_FSOffSw_enum"
  VAPM_FSOffSw_enum_Inproc/1 -> UnitConverter6/1
  UnitConverter6/1 -> VOUTP_FSOffSw_enum/1  "VOUTP_FSOffSw_enum"
  VAPM_FSOffSwTimeOut_flg/1 -> VAPM_FSOffSwTimeOut_flg_Inproc/1  "VAPM_FSOffSwTimeOut_flg"
  VAPM_FSOffSwTimeOut_flg_Inproc/1 -> UnitConverter7/1
  UnitConverter7/1 -> VOUTP_FSOffSwTimeOut_flg/1  "VOUTP_FSOffSwTimeOut_flg"
  VAPM_ChrgPlugSta_enum/1 -> VAPM_ChrgPlugSta_enum_Inproc/1  "VAPM_ChrgPlugSta_enum"
  VAPM_ChrgPlugSta_enum_Inproc/1 -> UnitConverter8/1
  UnitConverter8/1 -> VOUTP_ChrgPlugSta_enum/1  "VOUTP_ChrgPlugSta_enum"
  VAPM_PASDRMR_cm/1 -> VAPM_PASDRMR_cm_Inproc/1  "VAPM_PASDRMR_cm"
  VAPM_PASDRMR_cm_Inproc/1 -> UnitConverter9/1
  UnitConverter9/1 -> VOUTP_PASDRMR_cm/1  "VOUTP_PASDRMR_cm"
  VAPM_PASDRML_cm/1 -> VAPM_PASDRML_cm_Inproc/1  "VAPM_PASDRML_cm"
  VAPM_PASDRML_cm_Inproc/1 -> UnitConverter10/1
  UnitConverter10/1 -> VOUTP_PASDRML_cm/1  "VOUTP_PASDRML_cm"
  VAPM_PASDRCR_cm/1 -> VAPM_PASDRCR_cm_Inproc/1  "VAPM_PASDRCR_cm"
  VAPM_PASDRCR_cm_Inproc/1 -> UnitConverter11/1
  UnitConverter11/1 -> VOUTP_PASDRCR_cm/1  "VOUTP_PASDRCR_cm"
  VAPM_PASDRCL_cm/1 -> VAPM_PASDRCL_cm_Inproc/1  "VAPM_PASDRCL_cm"
  VAPM_PASDRCL_cm_Inproc/1 -> UnitConverter12/1
  UnitConverter12/1 -> VOUTP_PASDRCL_cm/1  "VOUTP_PASDRCL_cm"
  VAPM_PASDFMR_cm/1 -> VAPM_PASDFMR_cm_Inproc/1  "VAPM_PASDFMR_cm"
  VAPM_PASDFMR_cm_Inproc/1 -> UnitConverter13/1
  UnitConverter13/1 -> VOUTP_PASDFMR_cm/1  "VOUTP_PASDFMR_cm"
  VAPM_PASDFML_cm/1 -> VAPM_PASDFML_cm_Inproc/1  "VAPM_PASDFML_cm"
  VAPM_PASDFML_cm_Inproc/1 -> UnitConverter14/1
  UnitConverter14/1 -> VOUTP_PASDFML_cm/1  "VOUTP_PASDFML_cm"
  VAPM_PASDFCR_cm/1 -> VAPM_PASDFCR_cm_Inproc/1  "VAPM_PASDFCR_cm"
  VAPM_PASDFCR_cm_Inproc/1 -> UnitConverter15/1
  UnitConverter15/1 -> VOUTP_PASDFCR_cm/1  "VOUTP_PASDFCR_cm"
  VAPM_PASDFCL_cm/1 -> VAPM_PASDFCL_cm_Inproc/1  "VAPM_PASDFCL_cm"
  VAPM_PASDFCL_cm_Inproc/1 -> UnitConverter16/1
  UnitConverter16/1 -> VOUTP_PASDFCL_cm/1  "VOUTP_PASDFCL_cm"
  VAPM_APSDRLR_cm/1 -> VAPM_APSDRLR_cm_Inproc/1  "VAPM_APSDRLR_cm"
  VAPM_APSDRLR_cm_Inproc/1 -> UnitConverter17/1
  UnitConverter17/1 -> VOUTP_APSDRLR_cm/1  "VOUTP_APSDRLR_cm"
  VAPM_APSDRLL_cm/1 -> VAPM_APSDRLL_cm_Inproc/1  "VAPM_APSDRLL_cm"
  VAPM_APSDRLL_cm_Inproc/1 -> UnitConverter18/1
  UnitConverter18/1 -> VOUTP_APSDRLL_cm/1  "VOUTP_APSDRLL_cm"
  VAPM_APSDFLR_cm/1 -> VAPM_APSDFLR_cm_Inproc/1  "VAPM_APSDFLR_cm"
  VAPM_APSDFLR_cm_Inproc/1 -> UnitConverter19/1
  UnitConverter19/1 -> VOUTP_APSDFLR_cm/1  "VOUTP_APSDFLR_cm"
  VAPM_APSDFLL_cm/1 -> VAPM_APSDFLL_cm_Inproc/1  "VAPM_APSDFLL_cm"
  VAPM_APSDFLL_cm_Inproc/1 -> UnitConverter20/1
  UnitConverter20/1 -> VOUTP_APSDFLL_cm/1  "VOUTP_APSDFLL_cm"
  VAPM_PASAFCL_enum/1 -> VAPM_PASAFCL_enum_Inproc/1  "VAPM_PASAFCL_enum"
  VAPM_PASAFCL_enum_Inproc/1 -> UnitConverter21/1
  UnitConverter21/1 -> VOUTP_PASAFCL_enum/1  "VOUTP_PASAFCL_enum"
  VAPM_PASARMR_enum/1 -> VAPM_PASARMR_enum_Inproc/1  "VAPM_PASARMR_enum"
  VAPM_PASARMR_enum_Inproc/1 -> UnitConverter22/1
  UnitConverter22/1 -> VOUTP_PASARMR_enum/1  "VOUTP_PASARMR_enum"
  VAPM_PASARML_enum/1 -> VAPM_PASARML_enum_Inproc/1  "VAPM_PASARML_enum"
  VAPM_PASARML_enum_Inproc/1 -> UnitConverter23/1
  UnitConverter23/1 -> VOUTP_PASARML_enum/1  "VOUTP_PASARML_enum"
  VAPM_PASARCR_enum/1 -> VAPM_PASARCR_enum_Inproc/1  "VAPM_PASARCR_enum"
  VAPM_PASARCR_enum_Inproc/1 -> UnitConverter24/1
  UnitConverter24/1 -> VOUTP_PASARCR_enum/1  "VOUTP_PASARCR_enum"
  VAPM_PASARCL_enum/1 -> VAPM_PASARCL_enum_Inproc/1  "VAPM_PASARCL_enum"
  VAPM_PASARCL_enum_Inproc/1 -> UnitConverter25/1
  UnitConverter25/1 -> VOUTP_PASARCL_enum/1  "VOUTP_PASARCL_enum"
  VAPM_PASAFMR_enum/1 -> VAPM_PASAFMR_enum_Inproc/1  "VAPM_PASAFMR_enum"
  VAPM_PASAFMR_enum_Inproc/1 -> UnitConverter26/1
  UnitConverter26/1 -> VOUTP_PASAFMR_enum/1  "VOUTP_PASAFMR_enum"
  VAPM_PASAFML_enum/1 -> VAPM_PASAFML_enum_Inproc/1  "VAPM_PASAFML_enum"
  VAPM_PASAFML_enum_Inproc/1 -> UnitConverter27/1
  UnitConverter27/1 -> VOUTP_PASAFML_enum/1  "VOUTP_PASAFML_enum"
  VAPM_PASAFCR_enum/1 -> VAPM_PASAFCR_enum_Inproc/1  "VAPM_PASAFCR_enum"
  VAPM_PASAFCR_enum_Inproc/1 -> UnitConverter28/1
  UnitConverter28/1 -> VOUTP_PASAFCR_enum/1  "VOUTP_PASAFCR_enum"
  VAPM_USSStaRMR_flg/1 -> VAPM_USSStaRMR_flg_Inproc/1  "VAPM_USSStaRMR_flg"
  VAPM_USSStaRMR_flg_Inproc/1 -> UnitConverter29/1
  UnitConverter29/1 -> VOUTP_USSStaRMR_flg/1  "VOUTP_USSStaRMR_flg"
  VAPM_USSStaRML_flg/1 -> VAPM_USSStaRML_flg_Inproc/1  "VAPM_USSStaRML_flg"
  VAPM_USSStaRML_flg_Inproc/1 -> UnitConverter30/1
  UnitConverter30/1 -> VOUTP_USSStaRML_flg/1  "VOUTP_USSStaRML_flg"
  VAPM_USSStaRLR_flg/1 -> VAPM_USSStaRLR_flg_Inproc/1  "VAPM_USSStaRLR_flg"
  VAPM_USSStaRLR_flg_Inproc/1 -> UnitConverter31/1
  UnitConverter31/1 -> VOUTP_USSStaRLR_flg/1  "VOUTP_USSStaRLR_flg"
  VAPM_USSStaRLL_flg/1 -> VAPM_USSStaRLL_flg_Inproc/1  "VAPM_USSStaRLL_flg"
  VAPM_USSStaRLL_flg_Inproc/1 -> UnitConverter32/1
  UnitConverter32/1 -> VOUTP_USSStaRLL_flg/1  "VOUTP_USSStaRLL_flg"
  VAPM_USSStaRCR_flg/1 -> VAPM_USSStaRCR_flg_Inproc/1  "VAPM_USSStaRCR_flg"
  VAPM_USSStaRCR_flg_Inproc/1 -> UnitConverter33/1
  UnitConverter33/1 -> VOUTP_USSStaRCR_flg/1  "VOUTP_USSStaRCR_flg"
  VAPM_USSStaRCL_flg/1 -> VAPM_USSStaRCL_flg_Inproc/1  "VAPM_USSStaRCL_flg"
  VAPM_USSStaRCL_flg_Inproc/1 -> UnitConverter34/1
  UnitConverter34/1 -> VOUTP_USSStaRCL_flg/1  "VOUTP_USSStaRCL_flg"
  VAPM_USSStaFMR_flg/1 -> VAPM_USSStaFMR_flg_Inproc/1  "VAPM_USSStaFMR_flg"
  VAPM_USSStaFMR_flg_Inproc/1 -> UnitConverter35/1
  UnitConverter35/1 -> VOUTP_USSStaFMR_flg/1  "VOUTP_USSStaFMR_flg"
  VAPM_USSStaFML_flg/1 -> VAPM_USSStaFML_flg_Inproc/1  "VAPM_USSStaFML_flg"
  VAPM_USSStaFML_flg_Inproc/1 -> UnitConverter36/1
  UnitConverter36/1 -> VOUTP_USSStaFML_flg/1  "VOUTP_USSStaFML_flg"
  VAPM_USSStaFLR_flg/1 -> VAPM_USSStaFLR_flg_Inproc/1  "VAPM_USSStaFLR_flg"
  VAPM_USSStaFLR_flg_Inproc/1 -> UnitConverter37/1
  UnitConverter37/1 -> VOUTP_USSStaFLR_flg/1  "VOUTP_USSStaFLR_flg"
  VAPM_USSStaFLL_flg/1 -> VAPM_USSStaFLL_flg_Inproc/1  "VAPM_USSStaFLL_flg"
  VAPM_USSStaFLL_flg_Inproc/1 -> UnitConverter38/1
  UnitConverter38/1 -> VOUTP_USSStaFLL_flg/1  "VOUTP_USSStaFLL_flg"
  VAPM_USSStaFCR_flg/1 -> VAPM_USSStaFCR_flg_Inproc/1  "VAPM_USSStaFCR_flg"
  VAPM_USSStaFCR_flg_Inproc/1 -> UnitConverter39/1
  UnitConverter39/1 -> VOUTP_USSStaFCR_flg/1  "VOUTP_USSStaFCR_flg"
  VAPM_USSStaFCL_flg/1 -> VAPM_USSStaFCL_flg_Inproc/1  "VAPM_USSStaFCL_flg"
  VAPM_USSStaFCL_flg_Inproc/1 -> UnitConverter40/1
  UnitConverter40/1 -> VOUTP_USSStaFCL_flg/1  "VOUTP_USSStaFCL_flg"
  VAPM_Chime_enum/1 -> VAPM_Chime_enum_Inproc/1  "VAPM_Chime_enum"
  VAPM_Chime_enum_Inproc/1 -> UnitConverter41/1
  UnitConverter41/1 -> VOUTP_Chime_enum/1  "VOUTP_Chime_enum"
  VAPM_SNSRLayout_enum/1 -> VAPM_SNSRLayout_enum_Inproc/1  "VAPM_SNSRLayout_enum"
  VAPM_SNSRLayout_enum_Inproc/1 -> UnitConverter42/1
  UnitConverter42/1 -> VOUTP_SNSRLayout_enum/1  "VOUTP_SNSRLayout_enum"
  VAPM_StaFSya_flg/1 -> VAPM_StaFSya_flg_Inproc/1  "VAPM_StaFSya_flg"
  VAPM_StaFSya_flg_Inproc/1 -> UnitConverter43/1
  UnitConverter43/1 -> VOUTP_StaFSya_flg/1  "VOUTP_StaFSya_flg"
  VAPM_ModOperation_enum/1 -> VAPM_ModOperation_enum_Inproc/1  "VAPM_ModOperation_enum"
  VAPM_ModOperation_enum_Inproc/1 -> UnitConverter44/1
  UnitConverter44/1 -> VOUTP_ModOperation_enum/1  "VOUTP_ModOperation_enum"
  VAPM_BrkPedalPos_pct/1 -> VAPM_BrkPedalPos_pct_Inproc/1  "VAPM_BrkPedalPos_pct"
  VAPM_BrkPedalPos_pct_Inproc/1 -> UnitConverter45/1
  UnitConverter45/1 -> VOUTP_BrkPedalPos_pct/1  "VOUTP_BrkPedalPos_pct"
  VAPM_BrkPedalPosTimeOut_flg/1 -> VAPM_BrkPedalPosTimeOut_flg_Inproc/1  "VAPM_BrkPedalPosTimeOut_flg"
  VAPM_BrkPedalPosTimeOut_flg_Inproc/1 -> UnitConverter46/1
  UnitConverter46/1 -> VOUTP_BrkPedalPosTimeOut_flg/1  "VOUTP_BrkPedalPosTimeOut_flg"
  VAPM_LFRawWhlSpeed_kph/1 -> VAPM_LFRawWhlSpeed_kph_Inproc/1  "VAPM_LFRawWhlSpeed_kph"
  VAPM_LFRawWhlSpeed_kph_Inproc/1 -> UnitConverter47/1
  UnitConverter47/1 -> VOUTP_LFRawWhlSpeed_kph/1  "VOUTP_LFRawWhlSpeed_kph"
  VAPM_LFRawWhlSpeedTimeOut_flg/1 -> VAPM_LFRawWhlSpeedTimeOut_flg_Inproc/1  "VAPM_LFRawWhlSpeedTimeOut_flg"
  VAPM_LFRawWhlSpeedTimeOut_flg_Inproc/1 -> UnitConverter48/1
  UnitConverter48/1 -> VOUTP_LFRawWhlSpeedTimeOut_flg/1  "VOUTP_LFRawWhlSpeedTimeOut_flg"
  VAPM_RFRawWhlSpeed_kph/1 -> VAPM_RFRawWhlSpeed_kph_Inproc/1  "VAPM_RFRawWhlSpeed_kph"
  VAPM_RFRawWhlSpeed_kph_Inproc/1 -> UnitConverter49/1
  UnitConverter49/1 -> VOUTP_RFRawWhlSpeed_kph/1  "VOUTP_RFRawWhlSpeed_kph"
  VAPM_RFRawWhlSpeedTimeOut_flg/1 -> VAPM_RFRawWhlSpeedTimeOut_flg_Inproc/1  "VAPM_RFRawWhlSpeedTimeOut_flg"
  VAPM_RFRawWhlSpeedTimeOut_flg_Inproc/1 -> UnitConverter50/1
  UnitConverter50/1 -> VOUTP_RFRawWhlSpeedTimeOut_flg/1  "VOUTP_RFRawWhlSpeedTimeOut_flg"
  VAPM_LRRawWhlSpeed_kph/1 -> VAPM_LRRawWhlSpeed_kph_Inproc/1  "VAPM_LRRawWhlSpeed_kph"
  VAPM_LRRawWhlSpeed_kph_Inproc/1 -> UnitConverter51/1
  UnitConverter51/1 -> VOUTP_LRRawWhlSpeed_kph/1  "VOUTP_LRRawWhlSpeed_kph"
  VAPM_LRRawWhlSpeedTimeOut_flg/1 -> VAPM_LRRawWhlSpeedTimeOut_flg_Inproc/1  "VAPM_LRRawWhlSpeedTimeOut_flg"
  VAPM_LRRawWhlSpeedTimeOut_flg_Inproc/1 -> UnitConverter52/1
  UnitConverter52/1 -> VOUTP_LRRawWhlSpeedTimeOut_flg/1  "VOUTP_LRRawWhlSpeedTimeOut_flg"
  VAPM_RRRawWhlSpeed_kph/1 -> VAPM_RRRawWhlSpeed_kph_Inproc/1  "VAPM_RRRawWhlSpeed_kph"
  VAPM_RRRawWhlSpeed_kph_Inproc/1 -> UnitConverter53/1
  UnitConverter53/1 -> VOUTP_RRRawWhlSpeed_kph/1  "VOUTP_RRRawWhlSpeed_kph"
  VAPM_RRRawWhlSpeedTimeOut_flg/1 -> VAPM_RRRawWhlSpeedTimeOut_flg_Inproc/1  "VAPM_RRRawWhlSpeedTimeOut_flg"
  VAPM_RRRawWhlSpeedTimeOut_flg_Inproc/1 -> UnitConverter54/1
  UnitConverter54/1 -> VOUTP_RRRawWhlSpeedTimeOut_flg/1  "VOUTP_RRRawWhlSpeedTimeOut_flg"
  VAPM_LFRawWhlSpeedV_flg/1 -> VAPM_LFRawWhlSpeedV_flg_Inproc/1  "VAPM_LFRawWhlSpeedV_flg"
  VAPM_LFRawWhlSpeedV_flg_Inproc/1 -> UnitConverter55/1
  UnitConverter55/1 -> VOUTP_LFRawWhlSpeedV_flg/1  "VOUTP_LFRawWhlSpeedV_flg"
  VAPM_LFRawWhlSpeedVTimeOut_flg/1 -> VAPM_LFRawWhlSpeedVTimeOut_flg_Inproc/1  "VAPM_LFRawWhlSpeedVTimeOut_flg"
  VAPM_LFRawWhlSpeedVTimeOut_flg_Inproc/1 -> UnitConverter56/1
  UnitConverter56/1 -> VOUTP_LFRawWhlSpeedVTimeOut_flg/1  "VOUTP_LFRawWhlSpeedVTimeOut_flg"
  VAPM_RFRawWhlSpeedV_flg/1 -> VAPM_RFRawWhlSpeedV_flg_Inproc/1  "VAPM_RFRawWhlSpeedV_flg"
  VAPM_RFRawWhlSpeedV_flg_Inproc/1 -> UnitConverter57/1
  UnitConverter57/1 -> VOUTP_RFRawWhlSpeedV_flg/1  "VOUTP_RFRawWhlSpeedV_flg"
  VAPM_RFRawWhlSpeedVTimeOut_flg/1 -> VAPM_RFRawWhlSpeedVTimeOut_flg_Inproc/1  "VAPM_RFRawWhlSpeedVTimeOut_flg"
  VAPM_RFRawWhlSpeedVTimeOut_flg_Inproc/1 -> UnitConverter58/1
  UnitConverter58/1 -> VOUTP_RFRawWhlSpeedVTimeOut_flg/1  "VOUTP_RFRawWhlSpeedVTimeOut_flg"
  VAPM_LRRawWhlSpeedV_flg/1 -> VAPM_LRRawWhlSpeedV_flg_Inproc/1  "VAPM_LRRawWhlSpeedV_flg"
  VAPM_LRRawWhlSpeedV_flg_Inproc/1 -> UnitConverter59/1
  UnitConverter59/1 -> VOUTP_LRRawWhlSpeedV_flg/1  "VOUTP_LRRawWhlSpeedV_flg"
  VAPM_LRRawWhlSpeedVTimeOut_flg/1 -> VAPM_LRRawWhlSpeedVTimeOut_flg_Inproc/1  "VAPM_LRRawWhlSpeedVTimeOut_flg"
  VAPM_LRRawWhlSpeedVTimeOut_flg_Inproc/1 -> UnitConverter60/1
  UnitConverter60/1 -> VOUTP_LRRawWhlSpeedVTimeOut_flg/1  "VOUTP_LRRawWhlSpeedVTimeOut_flg"
  VAPM_RRRawWhlSpeedV_flg/1 -> VAPM_RRRawWhlSpeedV_flg_Inproc/1  "VAPM_RRRawWhlSpeedV_flg"
  VAPM_RRRawWhlSpeedV_flg_Inproc/1 -> UnitConverter61/1
  UnitConverter61/1 -> VOUTP_RRRawWhlSpeedV_flg/1  "VOUTP_RRRawWhlSpeedV_flg"
  VAPM_RRRawWhlSpeedVTimeOut_flg/1 -> VAPM_RRRawWhlSpeedVTimeOut_flg_Inproc/1  "VAPM_RRRawWhlSpeedVTimeOut_flg"
  VAPM_RRRawWhlSpeedVTimeOut_flg_Inproc/1 -> UnitConverter62/1
  UnitConverter62/1 -> VOUTP_RRRawWhlSpeedVTimeOut_flg/1  "VOUTP_RRRawWhlSpeedVTimeOut_flg"
  VAPM_LFWhlRotDir_enum/1 -> VAPM_LFWhlRotDir_enum_Inproc/1  "VAPM_LFWhlRotDir_enum"
  VAPM_LFWhlRotDir_enum_Inproc/1 -> UnitConverter63/1
  UnitConverter63/1 -> VOUTP_LFWhlRotDir_enum/1  "VOUTP_LFWhlRotDir_enum"
  VAPM_LFWhlRotDirTimeOut_flg/1 -> VAPM_LFWhlRotDirTimeOut_flg_Inproc/1  "VAPM_LFWhlRotDirTimeOut_flg"
  VAPM_LFWhlRotDirTimeOut_flg_Inproc/1 -> UnitConverter64/1
  UnitConverter64/1 -> VOUTP_LFWhlRotDirTimeOut_flg/1  "VOUTP_LFWhlRotDirTimeOut_flg"
  VAPM_RFWhlRotDir_enum/1 -> VAPM_RFWhlRotDir_enum_Inproc/1  "VAPM_RFWhlRotDir_enum"
  VAPM_RFWhlRotDir_enum_Inproc/1 -> UnitConverter65/1
  UnitConverter65/1 -> VOUTP_RFWhlRotDir_enum/1  "VOUTP_RFWhlRotDir_enum"
  VAPM_RFWhlRotDirTimeOut_flg/1 -> VAPM_RFWhlRotDirTimeOut_flg_Inproc/1  "VAPM_RFWhlRotDirTimeOut_flg"
  VAPM_RFWhlRotDirTimeOut_flg_Inproc/1 -> UnitConverter66/1
  UnitConverter66/1 -> VOUTP_RFWhlRotDirTimeOut_flg/1  "VOUTP_RFWhlRotDirTimeOut_flg"
  VAPM_LRWhlRotDir_enum/1 -> VAPM_LRWhlRotDir_enum_Inproc/1  "VAPM_LRWhlRotDir_enum"
  VAPM_LRWhlRotDir_enum_Inproc/1 -> UnitConverter67/1
  UnitConverter67/1 -> VOUTP_LRWhlRotDir_enum/1  "VOUTP_LRWhlRotDir_enum"
  VAPM_LRWhlRotDirTimeOut_flg/1 -> VAPM_LRWhlRotDirTimeOut_flg_Inproc/1  "VAPM_LRWhlRotDirTimeOut_flg"
  VAPM_LRWhlRotDirTimeOut_flg_Inproc/1 -> UnitConverter68/1
  UnitConverter68/1 -> VOUTP_LRWhlRotDirTimeOut_flg/1  "VOUTP_LRWhlRotDirTimeOut_flg"
  VAPM_RRWhlRotDir_enum/1 -> VAPM_RRWhlRotDir_enum_Inproc/1  "VAPM_RRWhlRotDir_enum"
  VAPM_RRWhlRotDir_enum_Inproc/1 -> UnitConverter69/1
  UnitConverter69/1 -> VOUTP_RRWhlRotDir_enum/1  "VOUTP_RRWhlRotDir_enum"
  VAPM_RRWhlRotDirTimeOut_flg/1 -> VAPM_RRWhlRotDirTimeOut_flg_Inproc/1  "VAPM_RRWhlRotDirTimeOut_flg"
  VAPM_RRWhlRotDirTimeOut_flg_Inproc/1 -> UnitConverter70/1
  UnitConverter70/1 -> VOUTP_RRWhlRotDirTimeOut_flg/1  "VOUTP_RRWhlRotDirTimeOut_flg"
  VAPM_LFPulseCountV_flg/1 -> VAPM_LFPulseCountV_flg_Inproc/1  "VAPM_LFPulseCountV_flg"
  VAPM_LFPulseCountV_flg_Inproc/1 -> UnitConverter71/1
  UnitConverter71/1 -> VOUTP_LFPulseCountV_flg/1  "VOUTP_LFPulseCountV_flg"
  VAPM_LFPulseCountVTimeOut_flg/1 -> VAPM_LFPulseCountVTimeOut_flg_Inproc/1  "VAPM_LFPulseCountVTimeOut_flg"
  VAPM_LFPulseCountVTimeOut_flg_Inproc/1 -> UnitConverter72/1
  UnitConverter72/1 -> VOUTP_LFPulseCountVTimeOut_flg/1  "VOUTP_LFPulseCountVTimeOut_flg"
  VAPM_RFPulseCountV_flg/1 -> VAPM_RFPulseCountV_flg_Inproc/1  "VAPM_RFPulseCountV_flg"
  VAPM_RFPulseCountV_flg_Inproc/1 -> UnitConverter73/1
  UnitConverter73/1 -> VOUTP_RFPulseCountV_flg/1  "VOUTP_RFPulseCountV_flg"
  VAPM_RFPulseCountVTimeOut_flg/1 -> VAPM_RFPulseCountVTimeOut_flg_Inproc/1  "VAPM_RFPulseCountVTimeOut_flg"
  VAPM_RFPulseCountVTimeOut_flg_Inproc/1 -> UnitConverter74/1
  UnitConverter74/1 -> VOUTP_RFPulseCountVTimeOut_flg/1  "VOUTP_RFPulseCountVTimeOut_flg"
  VAPM_LRPulseCountV_flg/1 -> VAPM_LRPulseCountV_flg_Inproc/1  "VAPM_LRPulseCountV_flg"
  VAPM_LRPulseCountV_flg_Inproc/1 -> UnitConverter75/1
  UnitConverter75/1 -> VOUTP_LRPulseCountV_flg/1  "VOUTP_LRPulseCountV_flg"
  VAPM_LRPulseCountVTimeOut_flg/1 -> VAPM_LRPulseCountVTimeOut_flg_Inproc/1  "VAPM_LRPulseCountVTimeOut_flg"
  VAPM_LRPulseCountVTimeOut_flg_Inproc/1 -> UnitConverter76/1
  UnitConverter76/1 -> VOUTP_LRPulseCountVTimeOut_flg/1  "VOUTP_LRPulseCountVTimeOut_flg"
  VAPM_RRPulseCountV_flg/1 -> VAPM_RRPulseCountV_flg_Inproc/1  "VAPM_RRPulseCountV_flg"
  VAPM_RRPulseCountV_flg_Inproc/1 -> UnitConverter77/1
  UnitConverter77/1 -> VOUTP_RRPulseCountV_flg/1  "VOUTP_RRPulseCountV_flg"
  VAPM_RRPulseCountVTimeOut_flg/1 -> VAPM_RRPulseCountVTimeOut_flg_Inproc/1  "VAPM_RRPulseCountVTimeOut_flg"
  VAPM_RRPulseCountVTimeOut_flg_Inproc/1 -> UnitConverter78/1
  UnitConverter78/1 -> VOUTP_RRPulseCountVTimeOut_flg/1  "VOUTP_RRPulseCountVTimeOut_flg"
  VAPM_LFPulseCount_enum/1 -> VAPM_LFPulseCount_enum_Inproc/1  "VAPM_LFPulseCount_enum"
  VAPM_LFPulseCount_enum_Inproc/1 -> UnitConverter79/1
  UnitConverter79/1 -> VOUTP_LFPulseCount_enum/1  "VOUTP_LFPulseCount_enum"
  VAPM_LFPulseCountTimeOut_flg/1 -> VAPM_LFPulseCountTimeOut_flg_Inproc/1  "VAPM_LFPulseCountTimeOut_flg"
  VAPM_LFPulseCountTimeOut_flg_Inproc/1 -> UnitConverter80/1
  UnitConverter80/1 -> VOUTP_LFPulseCountTimeOut_flg/1  "VOUTP_LFPulseCountTimeOut_flg"
  VAPM_RFPulseCount_enum/1 -> VAPM_RFPulseCount_enum_Inproc/1  "VAPM_RFPulseCount_enum"
  VAPM_RFPulseCount_enum_Inproc/1 -> UnitConverter81/1
  UnitConverter81/1 -> VOUTP_RFPulseCount_enum/1  "VOUTP_RFPulseCount_enum"
  VAPM_RFPulseCountTimeOut_flg/1 -> VAPM_RFPulseCountTimeOut_flg_Inproc/1  "VAPM_RFPulseCountTimeOut_flg"
  VAPM_RFPulseCountTimeOut_flg_Inproc/1 -> UnitConverter82/1
  UnitConverter82/1 -> VOUTP_RFPulseCountTimeOut_flg/1  "VOUTP_RFPulseCountTimeOut_flg"
  VAPM_LRPulseCount_enum/1 -> VAPM_LRPulseCount_enum_Inproc/1  "VAPM_LRPulseCount_enum"
  VAPM_LRPulseCount_enum_Inproc/1 -> UnitConverter83/1
  UnitConverter83/1 -> VOUTP_LRPulseCount_enum/1  "VOUTP_LRPulseCount_enum"
  VAPM_LRPulseCountTimeOut_flg/1 -> VAPM_LRPulseCountTimeOut_flg_Inproc/1  "VAPM_LRPulseCountTimeOut_flg"
  VAPM_LRPulseCountTimeOut_flg_Inproc/1 -> UnitConverter84/1
  UnitConverter84/1 -> VOUTP_LRPulseCountTimeOut_flg/1  "VOUTP_LRPulseCountTimeOut_flg"
  VAPM_RRPulseCount_enum/1 -> VAPM_RRPulseCount_enum_Inproc/1  "VAPM_RRPulseCount_enum"
  VAPM_RRPulseCount_enum_Inproc/1 -> UnitConverter85/1
  UnitConverter85/1 -> VOUTP_RRPulseCount_enum/1  "VOUTP_RRPulseCount_enum"
  VAPM_RRPulseCountTimeOut_flg/1 -> VAPM_RRPulseCountTimeOut_flg_Inproc/1  "VAPM_RRPulseCountTimeOut_flg"
  VAPM_RRPulseCountTimeOut_flg_Inproc/1 -> UnitConverter86/1
  UnitConverter86/1 -> VOUTP_RRPulseCountTimeOut_flg/1  "VOUTP_RRPulseCountTimeOut_flg"
  VAPM_ShifterHandleCmd_enum/1 -> VAPM_ShifterHandleCmd_enum_Inproc/1  "VAPM_ShifterHandleCmd_enum"
  VAPM_ShifterHandleCmd_enum_Inproc/1 -> UnitConverter87/1
  UnitConverter87/1 -> VOUTP_ShifterHandleCmd_enum/1  "VOUTP_ShifterHandleCmd_enum"
  VAPM_ShifterHandleCmdTimeOut_flg/1 -> VAPM_ShifterHandleCmdTimeOut_flg_Inproc/1  "VAPM_ShifterHandleCmdTimeOut_flg"
  VAPM_ShifterHandleCmdTimeOut_flg_Inproc/1 -> UnitConverter88/1
  UnitConverter88/1 -> VOUTP_ShifterHandleCmdTimeOut_flg/1  "VOUTP_ShifterHandleCmdTimeOut_flg"
  VAPM_DriIntend_enum/1 -> VAPM_DriIntend_enum_Inproc/1  "VAPM_DriIntend_enum"
  VAPM_DriIntend_enum_Inproc/1 -> UnitConverter89/1
  UnitConverter89/1 -> VOUTP_DriIntend_enum/1  "VOUTP_DriIntend_enum"
  VAPM_DriIntendTimeOut_flg/1 -> VAPM_DriIntendTimeOut_flg_Inproc/1  "VAPM_DriIntendTimeOut_flg"
  VAPM_DriIntendTimeOut_flg_Inproc/1 -> UnitConverter90/1
  UnitConverter90/1 -> VOUTP_DriIntendTimeOut_flg/1  "VOUTP_DriIntendTimeOut_flg"
  VAPM_EPSAOIControl_enum/1 -> VAPM_EPSAOIControl_enum_Inproc/1  "VAPM_EPSAOIControl_enum"
  VAPM_EPSAOIControl_enum_Inproc/1 -> UnitConverter91/1
  UnitConverter91/1 -> VOUTP_EPSAOIControl_enum/1  "VOUTP_EPSAOIControl_enum"
  VAPM_EPSAOIControlTimeOut_flg/1 -> VAPM_EPSAOIControlTimeOut_flg_Inproc/1  "VAPM_EPSAOIControlTimeOut_flg"
  VAPM_EPSAOIControlTimeOut_flg_Inproc/1 -> UnitConverter92/1
  UnitConverter92/1 -> VOUTP_EPSAOIControlTimeOut_flg/1  "VOUTP_EPSAOIControlTimeOut_flg"
  VAPM_SASAngle_Deg/1 -> VAPM_SASAngle_Deg_Inproc/1  "VAPM_SASAngle_Deg"
  VAPM_SASAngle_Deg_Inproc/1 -> UnitConverter93/1
  UnitConverter93/1 -> VOUTP_SASAngle_Deg/1  "VOUTP_SASAngle_Deg"
  VAPM_SASAngleTimeOut_flg/1 -> VAPM_SASAngleTimeOut_flg_Inproc/1  "VAPM_SASAngleTimeOut_flg"
  VAPM_SASAngleTimeOut_flg_Inproc/1 -> UnitConverter94/1
  UnitConverter94/1 -> VOUTP_SASAngleTimeOut_flg/1  "VOUTP_SASAngleTimeOut_flg"
  VAPM_SASSpeed_degps/1 -> VAPM_SASSpeed_degps_Inproc/1  "VAPM_SASSpeed_degps"
  VAPM_SASSpeed_degps_Inproc/1 -> UnitConverter95/1
  UnitConverter95/1 -> VOUTP_SASSpeed_degps/1  "VOUTP_SASSpeed_degps"
  VAPM_SASSpeedTimeOut_flg/1 -> VAPM_SASSpeedTimeOut_flg_Inproc/1  "VAPM_SASSpeedTimeOut_flg"
  VAPM_SASSpeedTimeOut_flg_Inproc/1 -> UnitConverter96/1
  UnitConverter96/1 -> VOUTP_SASSpeedTimeOut_flg/1  "VOUTP_SASSpeedTimeOut_flg"
  VAPM_SASSpeedValid_flg/1 -> VAPM_SASSpeedValid_flg_Inproc/1  "VAPM_SASSpeedValid_flg"
  VAPM_SASSpeedValid_flg_Inproc/1 -> UnitConverter97/1
  UnitConverter97/1 -> VOUTP_SASSpeedValid_flg/1  "VOUTP_SASSpeedValid_flg"
  VAPM_SASSpeedValidTimeOut_flg/1 -> VAPM_SASSpeedValidTimeOut_flg_Inproc/1  "VAPM_SASSpeedValidTimeOut_flg"
  VAPM_SASSpeedValidTimeOut_flg_Inproc/1 -> UnitConverter98/1
  UnitConverter98/1 -> VOUTP_SASSpeedValidTimeOut_flg/1  "VOUTP_SASSpeedValidTimeOut_flg"
  VAPM_SASCAL_flg/1 -> VAPM_SASCAL_flg_Inproc/1  "VAPM_SASCAL_flg"
  VAPM_SASCAL_flg_Inproc/1 -> UnitConverter99/1
  UnitConverter99/1 -> VOUTP_SASCAL_flg/1  "VOUTP_SASCAL_flg"
  VAPM_SASCALTimeOut_flg/1 -> VAPM_SASCALTimeOut_flg_Inproc/1  "VAPM_SASCALTimeOut_flg"
  VAPM_SASCALTimeOut_flg_Inproc/1 -> UnitConverter100/1
  UnitConverter100/1 -> VOUTP_SASCALTimeOut_flg/1  "VOUTP_SASCALTimeOut_flg"
  VAPM_SASV_flg/1 -> VAPM_SASV_flg_Inproc/1  "VAPM_SASV_flg"
  VAPM_SASV_flg_Inproc/1 -> UnitConverter101/1
  UnitConverter101/1 -> VOUTP_SASV_flg/1  "VOUTP_SASV_flg"
  VAPM_SASVTimeOut_flg/1 -> VAPM_SASVTimeOut_flg_Inproc/1  "VAPM_SASVTimeOut_flg"
  VAPM_SASVTimeOut_flg_Inproc/1 -> UnitConverter102/1
  UnitConverter102/1 -> VOUTP_SASVTimeOut_flg/1  "VOUTP_SASVTimeOut_flg"
  VAPM_GRADE_Deg/1 -> VAPM_GRADE_Deg_Inproc/1  "VAPM_GRADE_Deg"
  VAPM_GRADE_Deg_Inproc/1 -> UnitConverter103/1
  UnitConverter103/1 -> VOUTP_GRADE_Deg/1  "VOUTP_GRADE_Deg"
  VAPM_GRADETimeOut_flg/1 -> VAPM_GRADETimeOut_flg_Inproc/1  "VAPM_GRADETimeOut_flg"
  VAPM_GRADETimeOut_flg_Inproc/1 -> UnitConverter104/1
  UnitConverter104/1 -> VOUTP_GRADETimeOut_flg/1  "VOUTP_GRADETimeOut_flg"
  VAPM_YawRate_degps/1 -> VAPM_YawRate_degps_Inproc/1  "VAPM_YawRate_degps"
  VAPM_YawRate_degps_Inproc/1 -> UnitConverter105/1
  UnitConverter105/1 -> VOUTP_YawRate_degps/1  "VOUTP_YawRate_degps"
  VAPM_YawRateTimeOut_flg/1 -> VAPM_YawRateTimeOut_flg_Inproc/1  "VAPM_YawRateTimeOut_flg"
  VAPM_YawRateTimeOut_flg_Inproc/1 -> UnitConverter106/1
  UnitConverter106/1 -> VOUTP_YawRateTimeOut_flg/1  "VOUTP_YawRateTimeOut_flg"
  VAPM_LatAccel_Gps/1 -> VAPM_LatAccel_Gps_Inproc/1  "VAPM_LatAccel_Gps"
  VAPM_LatAccel_Gps_Inproc/1 -> UnitConverter107/1
  UnitConverter107/1 -> VOUTP_LatAccel_Gps/1  "VOUTP_LatAccel_Gps"
  VAPM_LatAccelTimeOut_flg/1 -> VAPM_LatAccelTimeOut_flg_Inproc/1  "VAPM_LatAccelTimeOut_flg"
  VAPM_LatAccelTimeOut_flg_Inproc/1 -> UnitConverter108/1
  UnitConverter108/1 -> VOUTP_LatAccelTimeOut_flg/1  "VOUTP_LatAccelTimeOut_flg"
  VAPM_LongAccel_Gps/1 -> VAPM_LongAccel_Gps_Inproc/1  "VAPM_LongAccel_Gps"
  VAPM_LongAccel_Gps_Inproc/1 -> UnitConverter109/1
  UnitConverter109/1 -> VOUTP_LongAccel_Gps/1  "VOUTP_LongAccel_Gps"
  VAPM_LongAccelTimeOut_flg/1 -> VAPM_LongAccelTimeOut_flg_Inproc/1  "VAPM_LongAccelTimeOut_flg"
  VAPM_LongAccelTimeOut_flg_Inproc/1 -> UnitConverter110/1
  UnitConverter110/1 -> VOUTP_LongAccelTimeOut_flg/1  "VOUTP_LongAccelTimeOut_flg"
  VAPM_MCPressure_bar/1 -> VAPM_MCPressure_bar_Inproc/1  "VAPM_MCPressure_bar"
  VAPM_MCPressure_bar_Inproc/1 -> UnitConverter111/1
  UnitConverter111/1 -> VOUTP_MCPressure_bar/1  "VOUTP_MCPressure_bar"
  VAPM_MCPressureTimeOut_flg/1 -> VAPM_MCPressureTimeOut_flg_Inproc/1  "VAPM_MCPressureTimeOut_flg"
  VAPM_MCPressureTimeOut_flg_Inproc/1 -> UnitConverter112/1
  UnitConverter112/1 -> VOUTP_MCPressureTimeOut_flg/1  "VOUTP_MCPressureTimeOut_flg"
  VAPM_YawRateV_flg/1 -> VAPM_YawRateV_flg_Inproc/1  "VAPM_YawRateV_flg"
  VAPM_YawRateV_flg_Inproc/1 -> UnitConverter113/1
  UnitConverter113/1 -> VOUTP_YawRateV_flg/1  "VOUTP_YawRateV_flg"
  VAPM_YawRateVTimeOut_flg/1 -> VAPM_YawRateVTimeOut_flg_Inproc/1  "VAPM_YawRateVTimeOut_flg"
  VAPM_YawRateVTimeOut_flg_Inproc/1 -> UnitConverter114/1
  UnitConverter114/1 -> VOUTP_YawRateVTimeOut_flg/1  "VOUTP_YawRateVTimeOut_flg"
  VAPM_LatAccelV_flg/1 -> VAPM_LatAccelV_flg_Inproc/1  "VAPM_LatAccelV_flg"
  VAPM_LatAccelV_flg_Inproc/1 -> UnitConverter115/1
